simulink model "ACC_Scenario_006_cs"  (R2014b)
settings: Solver=ode5  SolverMode=SingleTasking  StartTime=0.0  StopTime=inf  FixedStep=1/100  RelTol=1e-3
PreLoadFcn:
  | mbxruntime.callbacks.PreLoadFcn(bdroot);
  | check_NUTS_defined;
  | 
  | assignin('base',['model_closed_' bdroot],false);addpath('../includes_ACC');
PostLoadFcn:
  | mbxruntime.callbacks.PostLoadFcn(bdroot);
InitFcn:
  | mbxruntime.callbacks.InitFcn(bdroot);
StartFcn:
  | mbxruntime.callbacks.StartFcn(bdroot);
StopFcn:
  | mbxruntime.callbacks.StopFcn(bdroot);
model workspace: external: MAT-File .\ACC_Scenario_006_cs_hws.mat (data not in the file)
undefined symbols (not defined in the file or in its folder): mbxruntime, OrientationPitch, OrientationRoll, PositionX, PositionY, PositionZ, tabledata, warningInitialVelocity, x0
undefined symbols (not defined in the file): ACC_Scenario_006_cs_061450488d6753c4, ACC_Scenario_006_cs_13896134c615b72a, ACC_Scenario_006_cs_18eaf2a52f2ef75d, ACC_Scenario_006_cs_59e375456829d2f0, ACC_Scenario_006_cs_8a2109b915871f11, ACC_Scenario_006_cs_a4f79cab717c06e2, ACC_Scenario_006_cs_Audi_A8_1_Dynamics_Simple_initialPitch, ACC_Scenario_006_cs_Audi_A8_1_Dynamics_Simple_initialRoll, ACC_Scenario_006_cs_Audi_A8_1_Dynamics_Simple_initialX, ACC_Scenario_006_cs_Audi_A8_1_Dynamics_Simple_initialY, ACC_Scenario_006_cs_Audi_A8_1_Dynamics_Simple_initialYaw, ACC_Scenario_006_cs_Audi_A8_1_Dynamics_Simple_initialZ, ACC_Scenario_006_cs_BMW_X5_1_Path_pathUniqueID, ACC_Scenario_006_cs_BMW_X5_1_SpeedProfile_speedProfileUniqueID, ACC_Scenario_006_cs_e4633c18fd34a832, ACC_Scenario_006_cs_f83c81dc10cd364a, ACC_Scenario_006_cs_Fiat_Bravo_1_Path_pathUniqueID, ACC_Scenario_006_cs_Ford_Fiesta_1_Path_pathUniqueID, ACC_Scenario_006_cs_Honda_Pan_European_1_Path_pathUniqueID, ACC_Scenario_006_cs_Mazda_RX8_1_Path_pathUniqueID, ACC_Scenario_006_cs_Sphere_1_Dynamics_Empty_STATE_Sphere_1_x0, ACC_Scenario_006_cs_Sphere_1_Dynamics_Empty_STATE_Sphere_1_y0, ACC_Scenario_006_cs_Sphere_1_Dynamics_Empty_STATE_Sphere_1_Yaw0, ACC_Scenario_006_cs_Sphere_1_Dynamics_Empty_STATE_Sphere_1_z0, ACC_Scenario_006_cs_Toyota_Yaris_1_Path_pathUniqueID, SteeringColumn, SteeringWheel, Wheel0, Wheel0_Suspension, Wheel1, Wheel1_Suspension, WheelL0, WheelL1, WheelR0, WheelR1
libraries: simulink_extras x60, simulink x21, PreScanSimulinkLibrary x5, PreScanUsefulBlocks x2
(part 1 of 24)
CloseFcn:
  | mbxruntime.callbacks.CloseFcn(bdroot);
  | evalin('base',['clear model_closed_' bdroot]);
settings Model: Creator=PRESCAN  LastModifiedBy=jenkins
settings DataIOCC: SignalLoggingSaveFormat=ModelDataLogs
settings OptimizationCC: InlineParams=on  ExpressionDepthLimit=2147483647  InitFltsAndDblsToZero=on
settings DebuggingCC: SaveWithParameterizedLinksMsg=none  UnderspecifiedInitializationDetection=Classic  MergeDetectMultiDrivingBlocksExec=none  SignalResolutionControl=TryResolveAllWithWarning  SolverPrmCheckMsg=none  MultiTaskDSMMsg=warning  MultiTaskCondExecSysMsg=none  FcnCallInpInsideContextMsg=UseLocalSettings  StateNameClashWarn=warning
settings ModelReferenceCC: UpdateModelReferenceTargets=IfOutOfDate
settings SFSimCC: SimParseCustomCode=off
settings SFSimCC: SimCustomHeaderCode=|
  | #include "prescan.h"
  | #include "prescan_platform.h"
settings RTWCC: IncludeERTFirstTime=on
settings GRTTargetCC: TargetFcnLib=ansi_tfl_tmw.mat  CombineOutputUpdateFcns=off  GRTInterface=on

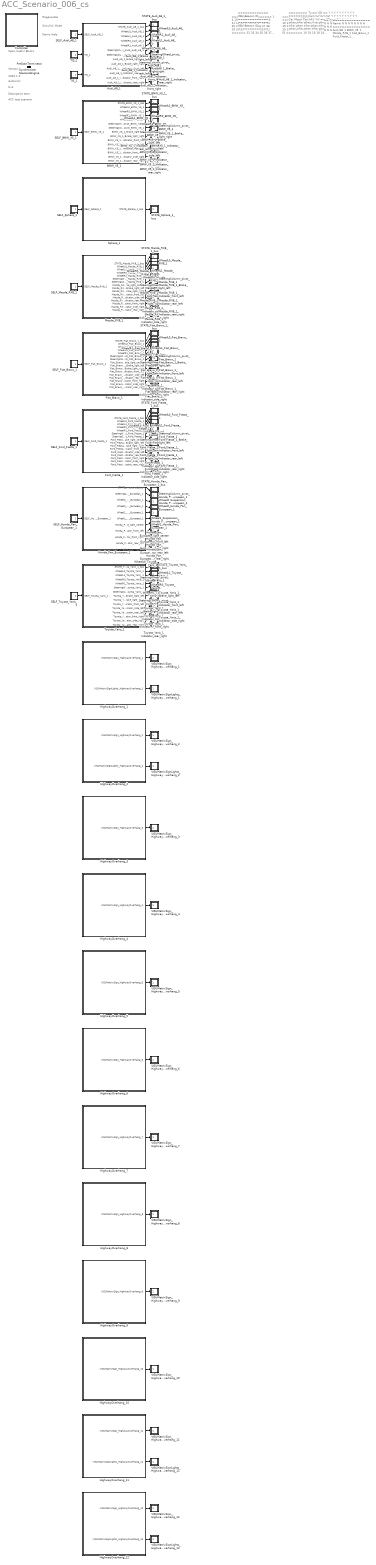
== system ACC_Scenario_006_cs ==
  note: Regenerate
  note: Simulink Mode
  note: Open Useful Blocks
  note: 2020.1.0
  note: Version:
  note: Author(s):
  note: N.A.
  note: Descriptive text:
  note: ACC test scenario
  note: Demo Help
  note: ======
      | Num ID
      | ======
      | 1
      | 4
      | 102
      | 231
      | 232
      | 233
      | 234
      | 8
      | 10
      | 11
      | 12
      | 13
      | 14
      | 15
      | 16
      | 17
      | 18
      | 19
      | 20
      | 21
      | 22
      | 23
      | 24
      | 25
      | 26
      | 27
      | 28
      | 29
      | 30
      | 31
      | ======
      | Num ID
      | ======
      | 32
      | 33
      | 34
      | 35
      | 36
      | 37
      | 38
      | 39
  note: =============
      | OBU-Beacon ID
      | =============
      |
      |
      |
      |
      |
      |
      |
      |
      |
      |
      |
      |
      |
      |
      |
      |
      |
      |
      |
      |
      |
      |
      |
      |
      |
      |
      |
      |
      |
      |
      | =============
      | OBU-Beacon ID
      | =============
  note: =======
      | Type ID
      | =======
      | 1
      | 1
      | 1
      | 1
      | 1
      | 2
      | 1
      | 19
      | 19
      | 19
      | 19
      | 19
      | 19
      | 19
      | 19
      | 19
      | 19
      | 19
      | 19
      | 19
      | 19
      | 19
      | 19
      | 19
      | 19
      | 19
      | 19
      | 19
      | 19
      | 19
      | =======
      | Type ID
      | =======
      | 19
      | 19
      | 19
      | 19
      | 19
      | 19
      | 19
      | 19
  note: ========
      | Type Tag
      | ========
      | Car
      | Car
      | Car
      | Car
      | Car
      | Motor
      | Car
      | Infra other
      | Infra other
      | Infra other
      | Infra other
      | Infra other
      | Infra other
      | Infra other
      | Infra other
      | Infra other
      | Infra other
      | Infra other
      | Infra other
      | Infra other
      | Infra other
      | Infra other
      | Infra other
      | Infra other
      | Infra other
      | Infra other
      | Infra other
      | Infra other
      | Infra other
      | Infra other
      | ========
      | Type Tag
      | ========
      | Infra other
      | Infra other
      | Infra other
      | Infra other
      | Infra other
      | Infra other
      | Infra other
      | Infra other
  note: ==
      | SD
      | ==
      | Y
      | Y
      | Y
      | Y
      | Y
      | Y
      | Y
      | Y
      | Y
      | Y
      | Y
      | Y
      | Y
      | Y
      | Y
      | Y
      | Y
      | Y
      | Y
      | Y
      | Y
      | Y
      | Y
      | Y
      | Y
      | Y
      | Y
      | Y
      | Y
      | Y
      | ==
      | SD
      | ==
      | Y
      | Y
      | Y
      | Y
      | Y
      | Y
      | Y
      | Y
  note: ==
      | CD
      | ==
      | N
      | N
      | N
      | N
      | N
      | N
      | N
      | N
      | N
      | N
      | N
      | N
      | N
      | N
      | N
      | N
      | N
      | N
      | N
      | N
      | N
      | N
      | N
      | N
      | N
      | N
      | N
      | N
      | N
      | N
      | ==
      | CD
      | ==
      | N
      | N
      | N
      | N
      | N
      | N
      | N
      | N
  note: ================
      | Name
      | ================
      | Audi_A8_1
      | BMW_X5_1
      | Mazda_RX8_1
      | Fiat_Bravo_1
      | Ford_Fiesta_1
      | Honda_Pan_European_1
      | Toyota_Yaris_1
      | ReflectorSign_1
      | ReflectorSign_2
      | ReflectorSign_3
      | ReflectorSign_4
      | ReflectorSign_5
      | ReflectorSign_6
      | ReflectorSign_7
      | ReflectorSign_8
      | ReflectorSign_9
      | ReflectorSign_10
      | ReflectorSign_11
      | ReflectorSign_12
      | ReflectorSign_13
      | ReflectorSign_14
      | ReflectorSign_15
      | ReflectorSign_16
      | ReflectorSign_17
      | ReflectorSign_18
      | ReflectorSign_19
      | ReflectorSign_20
      | ReflectorSign_21
      | ReflectorSign_22
      | ReflectorSign_23
      | ================
      | Name
      | ================
      | ReflectorSign_24
      | ReflectorSign_25
      | ReflectorSign_26
      | ReflectorSign_27
      | ReflectorSign_28
      | ReflectorSign_29
      | ReflectorSign_30
      | ReflectorSign_31
  Audi_A8_1 : Subsystem  Tag=WorldObjectSubSystem  InitFcn=UniqueId = '16';
      mask init:
      | modelPath = GenericModelHelper.getGenericModelFilePath('ModelDepo','Vehicles\Audi_A8\Audi_A8.pgmb','e33fe1ddcf3e8ae97caccbc8f2fa74ac');imagePath = GenericModelHelper.getCompilationPicture(modelPath, 'Audi_A8_HighPoly.png');
      mask Display: image(imread(imagePath));color('white');text(0, 0, ' ID=1\n')
  Audi_A8_1_Brake_light_left : Subsystem  Tag=actuator/BrakeLightL  Priority=0  LoadFcn=load('PreScanVisuLightActuatorData');load('PrescanRPYData');load('PrescanXYZData');load('PreScanRGBData')  mask(PreScan Sink Block: VisuActiveLight){}
      mask help:
      | The VisuActiveLight block provides a way for detailed animation of Light Sources, such as the indicator, brake, fog and main lights of a vehicle, or a light post.
      |
      | For more information, please click Help.
      settings: OpenFcn=open_system([gcb '/Actuator'],'mask')
      mask Help: eval('openHelp(209)')
      mask Display: image(imread('HeadLight.png'))
  Audi_A8_1_Brake_light_right : Subsystem  Tag=actuator/BrakeLightR  Priority=0  LoadFcn=load('PreScanVisuLightActuatorData');load('PrescanRPYData');load('PrescanXYZData');load('PreScanRGBData')  mask(PreScan Sink Block: VisuActiveLight){}
      mask help:
      | The VisuActiveLight block provides a way for detailed animation of Light Sources, such as the indicator, brake, fog and main lights of a vehicle, or a light post.
      |
      | For more information, please click Help.
      settings: OpenFcn=open_system([gcb '/Actuator'],'mask')
      mask Help: eval('openHelp(209)')
      mask Display: image(imread('HeadLight.png'))
  Audi_A8_1_Indicator_front_left : Subsystem  Tag=actuator/IndicatorFL  Priority=0  LoadFcn=load('PreScanVisuLightActuatorData');load('PrescanRPYData');load('PrescanXYZData');load('PreScanRGBData')  mask(PreScan Sink Block: VisuActiveLight){}
      mask help:
      | The VisuActiveLight block provides a way for detailed animation of Light Sources, such as the indicator, brake, fog and main lights of a vehicle, or a light post.
      |
      | For more information, please click Help.
      settings: OpenFcn=open_system([gcb '/Actuator'],'mask')
      mask Help: eval('openHelp(209)')
      mask Display: image(imread('HeadLight.png'))
  Audi_A8_1_Indicator_front_right : Subsystem  Tag=actuator/IndicatorFR  Priority=0  LoadFcn=load('PreScanVisuLightActuatorData');load('PrescanRPYData');load('PrescanXYZData');load('PreScanRGBData')  mask(PreScan Sink Block: VisuActiveLight){}
      mask help:
      | The VisuActiveLight block provides a way for detailed animation of Light Sources, such as the indicator, brake, fog and main lights of a vehicle, or a light post.
      |
      | For more information, please click Help.
      settings: OpenFcn=open_system([gcb '/Actuator'],'mask')
      mask Help: eval('openHelp(209)')
      mask Display: image(imread('HeadLight.png'))
  Audi_A8_1_Indicator_rear_left : Subsystem  Tag=actuator/IndicatorRL  Priority=0  LoadFcn=load('PreScanVisuLightActuatorData');load('PrescanRPYData');load('PrescanXYZData');load('PreScanRGBData')  mask(PreScan Sink Block: VisuActiveLight){}
      mask help:
      | The VisuActiveLight block provides a way for detailed animation of Light Sources, such as the indicator, brake, fog and main lights of a vehicle, or a light post.
      |
      | For more information, please click Help.
      settings: OpenFcn=open_system([gcb '/Actuator'],'mask')
      mask Help: eval('openHelp(209)')
      mask Display: image(imread('HeadLight.png'))
  Audi_A8_1_Indicator_rear_right : Subsystem  Tag=actuator/IndicatorRR  Priority=0  LoadFcn=load('PreScanVisuLightActuatorData');load('PrescanRPYData');load('PrescanXYZData');load('PreScanRGBData')  mask(PreScan Sink Block: VisuActiveLight){}
      mask help:
      | The VisuActiveLight block provides a way for detailed animation of Light Sources, such as the indicator, brake, fog and main lights of a vehicle, or a light post.
      |
      | For more information, please click Help.
      settings: OpenFcn=open_system([gcb '/Actuator'],'mask')
      mask Help: eval('openHelp(209)')
      mask Display: image(imread('HeadLight.png'))
  BMW_X5_1 : Subsystem  Tag=WorldObjectSubSystem  InitFcn=UniqueId = '21';
      mask init:
      | modelPath = GenericModelHelper.getGenericModelFilePath('ModelDepo','Vehicles\BMW_X5\BMW_X5.pgmb','bfeb1c11467705ab888b3011684c848b');imagePath = GenericModelHelper.getCompilationPicture(modelPath, 'BMW_X5_HighPoly.png');
      mask Display: image(imread(imagePath));color('white');text(0, 0, ' ID=4\n')
  BMW_X5_1_Brake_light_left : Subsystem  Tag=actuator/BrakeLightL  Priority=0  LoadFcn=load('PreScanVisuLightActuatorData');load('PrescanRPYData');load('PrescanXYZData');load('PreScanRGBData')  mask(PreScan Sink Block: VisuActiveLight){}
      mask help:
      | The VisuActiveLight block provides a way for detailed animation of Light Sources, such as the indicator, brake, fog and main lights of a vehicle, or a light post.
      |
      | For more information, please click Help.
      settings: OpenFcn=open_system([gcb '/Actuator'],'mask')
      mask Help: eval('openHelp(209)')
      mask Display: image(imread('HeadLight.png'))
  BMW_X5_1_Brake_light_right : Subsystem  Tag=actuator/BrakeLightR  Priority=0  LoadFcn=load('PreScanVisuLightActuatorData');load('PrescanRPYData');load('PrescanXYZData');load('PreScanRGBData')  mask(PreScan Sink Block: VisuActiveLight){}
      mask help:
      | The VisuActiveLight block provides a way for detailed animation of Light Sources, such as the indicator, brake, fog and main lights of a vehicle, or a light post.
      |
      | For more information, please click Help.
      settings: OpenFcn=open_system([gcb '/Actuator'],'mask')
      mask Help: eval('openHelp(209)')
      mask Display: image(imread('HeadLight.png'))
  BMW_X5_1_Indicator_front_left : Subsystem  Tag=actuator/IndicatorFL  Priority=0  LoadFcn=load('PreScanVisuLightActuatorData');load('PrescanRPYData');load('PrescanXYZData');load('PreScanRGBData')  mask(PreScan Sink Block: VisuActiveLight){}
      mask help:
      | The VisuActiveLight block provides a way for detailed animation of Light Sources, such as the indicator, brake, fog and main lights of a vehicle, or a light post.
      |
      | For more information, please click Help.
      settings: OpenFcn=open_system([gcb '/Actuator'],'mask')
      mask Help: eval('openHelp(209)')
      mask Display: image(imread('HeadLight.png'))
  BMW_X5_1_Indicator_front_right : Subsystem  Tag=actuator/IndicatorFR  Priority=0  LoadFcn=load('PreScanVisuLightActuatorData');load('PrescanRPYData');load('PrescanXYZData');load('PreScanRGBData')  mask(PreScan Sink Block: VisuActiveLight){}
      mask help:
      | The VisuActiveLight block provides a way for detailed animation of Light Sources, such as the indicator, brake, fog and main lights of a vehicle, or a light post.
      |
      | For more information, please click Help.
      settings: OpenFcn=open_system([gcb '/Actuator'],'mask')
      mask Help: eval('openHelp(209)')
      mask Display: image(imread('HeadLight.png'))
  BMW_X5_1_Indicator_rear_left : Subsystem  Tag=actuator/IndicatorRL  Priority=0  LoadFcn=load('PreScanVisuLightActuatorData');load('PrescanRPYData');load('PrescanXYZData');load('PreScanRGBData')  mask(PreScan Sink Block: VisuActiveLight){}
      mask help:
      | The VisuActiveLight block provides a way for detailed animation of Light Sources, such as the indicator, brake, fog and main lights of a vehicle, or a light post.
      |
      | For more information, please click Help.
      settings: OpenFcn=open_system([gcb '/Actuator'],'mask')
      mask Help: eval('openHelp(209)')
      mask Display: image(imread('HeadLight.png'))
  BMW_X5_1_Indicator_rear_right : Subsystem  Tag=actuator/IndicatorRR  Priority=0  LoadFcn=load('PreScanVisuLightActuatorData');load('PrescanRPYData');load('PrescanXYZData');load('PreScanRGBData')  mask(PreScan Sink Block: VisuActiveLight){}
      mask help:
      | The VisuActiveLight block provides a way for detailed animation of Light Sources, such as the indicator, brake, fog and main lights of a vehicle, or a light post.
      |
      | For more information, please click Help.
      settings: OpenFcn=open_system([gcb '/Actuator'],'mask')
      mask Help: eval('openHelp(209)')
      mask Display: image(imread('HeadLight.png'))
  BMW_X5_1_Indicator_side_left : Subsystem  Tag=actuator/IndicatorSL  Priority=0  LoadFcn=load('PreScanVisuLightActuatorData');load('PrescanRPYData');load('PrescanXYZData');load('PreScanRGBData')  mask(PreScan Sink Block: VisuActiveLight){}
      mask help:
      | The VisuActiveLight block provides a way for detailed animation of Light Sources, such as the indicator, brake, fog and main lights of a vehicle, or a light post.
      |
      | For more information, please click Help.
      settings: OpenFcn=open_system([gcb '/Actuator'],'mask')
      mask Help: eval('openHelp(209)')
      mask Display: image(imread('HeadLight.png'))
  BMW_X5_1_Indicator_side_right : Subsystem  Tag=actuator/IndicatorSR  Priority=0  LoadFcn=load('PreScanVisuLightActuatorData');load('PrescanRPYData');load('PrescanXYZData');load('PreScanRGBData')  mask(PreScan Sink Block: VisuActiveLight){}
      mask help:
      | The VisuActiveLight block provides a way for detailed animation of Light Sources, such as the indicator, brake, fog and main lights of a vehicle, or a light post.
      |
      | For more information, please click Help.
      settings: OpenFcn=open_system([gcb '/Actuator'],'mask')
      mask Help: eval('openHelp(209)')
      mask Display: image(imread('HeadLight.png'))
  Controller : Subsystem  Description=8A3CD2955739A82C886C20AE3E253D78460D53180EE2C1B14CC08DF75A70BE77  Priority=-1  LoadFcn=load PreScanControllerData  mask(PreScan Simulation Controller){prescanversion='2020.1.0', ModelReferencing=off, TimeStep=1/100, ControlMode=0, PreScanExecutionMode=on, ControllerCount=0, ControllerIndex=0, ControllerOptions=''}
      mask prompts: prescanversion "PreScan Version"; ModelReferencing "Use Model Referencing"; TimeStep "Upload Period [s]"; ControlMode "Control Mode"; PreScanExecutionMode "Execution Mode"; ControllerCount "Controller Count"; ControllerIndex "Controller Index"; ControllerOptions "Controller Options"
      mask help:
      | Please do not remove this block from the compilation sheet,
      | as it connects the model to the PreScan environment.
      mask init:
      | model = bdroot(gcb);
      | ExperimentFile = mbxruntime.findExperimentFile(model,true); %relative path
      | 
      | [d1, d2, d3, prescandata] = prescan_Settings();
      | ModelDepo = fullfile(prescandata,'ModelDepo'); 
      | 
      | RTmode = mbxruntime.getRTMode(model);
      | 
      | SimulationMode = get_param(bdroot,'SimulationMode');
      | if strcmp(SimulationMode, 'rapid-accelerator')
      |     SimulationMode = 'external';
      | end
      | TargetName = get_param(bdroot,'SystemTargetFile');
      settings: ModelCloseFcn=assignin('base',['model_closed_' bdroot],true);
      mask Help: eval('openHelp(812)')
      mask Display: image(imread('prescanlogo.ico'))
  Fiat_Bravo_1 : Subsystem  Tag=WorldObjectSubSystem  InitFcn=UniqueId = '350';
      mask init:
      | modelPath = GenericModelHelper.getGenericModelFilePath('ModelDepo','Vehicles\Fiat_Bravo\Fiat_Bravo.pgmb','a97eb0ec4093646e5d079d2ab9a2eab7');imagePath = GenericModelHelper.getCompilationPicture(modelPath, 'Fiat_Bravo_HighPoly.png');
      mask Display: image(imread(imagePath));color('white');text(0, 0, ' ID=231\n')
  Fiat_Bravo_1_Brake_light_center : Subsystem  Tag=actuator/BrakeLightM  Priority=0  LoadFcn=load('PreScanVisuLightActuatorData');load('PrescanRPYData');load('PrescanXYZData');load('PreScanRGBData')  mask(PreScan Sink Block: VisuActiveLight){}
      mask help:
      | The VisuActiveLight block provides a way for detailed animation of Light Sources, such as the indicator, brake, fog and main lights of a vehicle, or a light post.
      |
      | For more information, please click Help.
      settings: OpenFcn=open_system([gcb '/Actuator'],'mask')
      mask Help: eval('openHelp(209)')
      mask Display: image(imread('HeadLight.png'))
  Fiat_Bravo_1_Brake_light_left : Subsystem  Tag=actuator/BrakeLightL  Priority=0  LoadFcn=load('PreScanVisuLightActuatorData');load('PrescanRPYData');load('PrescanXYZData');load('PreScanRGBData')  mask(PreScan Sink Block: VisuActiveLight){}
      mask help:
      | The VisuActiveLight block provides a way for detailed animation of Light Sources, such as the indicator, brake, fog and main lights of a vehicle, or a light post.
      |
      | For more information, please click Help.
      settings: OpenFcn=open_system([gcb '/Actuator'],'mask')
      mask Help: eval('openHelp(209)')
      mask Display: image(imread('HeadLight.png'))
  Fiat_Bravo_1_Brake_light_right : Subsystem  Tag=actuator/BrakeLightR  Priority=0  LoadFcn=load('PreScanVisuLightActuatorData');load('PrescanRPYData');load('PrescanXYZData');load('PreScanRGBData')  mask(PreScan Sink Block: VisuActiveLight){}
      mask help:
      | The VisuActiveLight block provides a way for detailed animation of Light Sources, such as the indicator, brake, fog and main lights of a vehicle, or a light post.
      |
      | For more information, please click Help.
      settings: OpenFcn=open_system([gcb '/Actuator'],'mask')
      mask Help: eval('openHelp(209)')
      mask Display: image(imread('HeadLight.png'))
  Fiat_Bravo_1_Indicator_front_left : Subsystem  Tag=actuator/IndicatorFL  Priority=0  LoadFcn=load('PreScanVisuLightActuatorData');load('PrescanRPYData');load('PrescanXYZData');load('PreScanRGBData')  mask(PreScan Sink Block: VisuActiveLight){}
      mask help:
      | The VisuActiveLight block provides a way for detailed animation of Light Sources, such as the indicator, brake, fog and main lights of a vehicle, or a light post.
      |
      | For more information, please click Help.
      settings: OpenFcn=open_system([gcb '/Actuator'],'mask')
      mask Help: eval('openHelp(209)')
      mask Display: image(imread('HeadLight.png'))
  Fiat_Bravo_1_Indicator_front_right : Subsystem  Tag=actuator/IndicatorFR  Priority=0  LoadFcn=load('PreScanVisuLightActuatorData');load('PrescanRPYData');load('PrescanXYZData');load('PreScanRGBData')  mask(PreScan Sink Block: VisuActiveLight){}
      mask help:
      | The VisuActiveLight block provides a way for detailed animation of Light Sources, such as the indicator, brake, fog and main lights of a vehicle, or a light post.
      |
      | For more information, please click Help.
      settings: OpenFcn=open_system([gcb '/Actuator'],'mask')
      mask Help: eval('openHelp(209)')
      mask Display: image(imread('HeadLight.png'))
  Fiat_Bravo_1_Indicator_rear_left : Subsystem  Tag=actuator/IndicatorRL  Priority=0  LoadFcn=load('PreScanVisuLightActuatorData');load('PrescanRPYData');load('PrescanXYZData');load('PreScanRGBData')  mask(PreScan Sink Block: VisuActiveLight){}
      mask help:
      | The VisuActiveLight block provides a way for detailed animation of Light Sources, such as the indicator, brake, fog and main lights of a vehicle, or a light post.
      |
      | For more information, please click Help.
      settings: OpenFcn=open_system([gcb '/Actuator'],'mask')
      mask Help: eval('openHelp(209)')
      mask Display: image(imread('HeadLight.png'))
  Fiat_Bravo_1_Indicator_rear_right : Subsystem  Tag=actuator/IndicatorRR  Priority=0  LoadFcn=load('PreScanVisuLightActuatorData');load('PrescanRPYData');load('PrescanXYZData');load('PreScanRGBData')  mask(PreScan Sink Block: VisuActiveLight){}
      mask help:
      | The VisuActiveLight block provides a way for detailed animation of Light Sources, such as the indicator, brake, fog and main lights of a vehicle, or a light post.
      |
      | For more information, please click Help.
      settings: OpenFcn=open_system([gcb '/Actuator'],'mask')
      mask Help: eval('openHelp(209)')
      mask Display: image(imread('HeadLight.png'))
  Fiat_Bravo_1_Indicator_side_left : Subsystem  Tag=actuator/IndicatorSL  Priority=0  LoadFcn=load('PreScanVisuLightActuatorData');load('PrescanRPYData');load('PrescanXYZData');load('PreScanRGBData')  mask(PreScan Sink Block: VisuActiveLight){}
      mask help:
      | The VisuActiveLight block provides a way for detailed animation of Light Sources, such as the indicator, brake, fog and main lights of a vehicle, or a light post.
      |
      | For more information, please click Help.
      settings: OpenFcn=open_system([gcb '/Actuator'],'mask')
      mask Help: eval('openHelp(209)')
      mask Display: image(imread('HeadLight.png'))
  Fiat_Bravo_1_Indicator_side_right : Subsystem  Tag=actuator/IndicatorSR  Priority=0  LoadFcn=load('PreScanVisuLightActuatorData');load('PrescanRPYData');load('PrescanXYZData');load('PreScanRGBData')  mask(PreScan Sink Block: VisuActiveLight){}
      mask help:
      | The VisuActiveLight block provides a way for detailed animation of Light Sources, such as the indicator, brake, fog and main lights of a vehicle, or a light post.
      |
      | For more information, please click Help.
      settings: OpenFcn=open_system([gcb '/Actuator'],'mask')
      mask Help: eval('openHelp(209)')
      mask Display: image(imread('HeadLight.png'))
  Ford_Fiesta_1 : Subsystem  Tag=WorldObjectSubSystem  InitFcn=UniqueId = '353';
      mask init:
      | modelPath = GenericModelHelper.getGenericModelFilePath('ModelDepo','Vehicles\Ford_Fiesta\Ford_Fiesta.pgmb','fe2c7a73e0a60cba76689b71cd1bb76a');imagePath = GenericModelHelper.getCompilationPicture(modelPath, 'Ford_Fiesta_HighPoly.png');
      mask Display: image(imread(imagePath));color('white');text(0, 0, ' ID=232\n')
  Ford_Fiesta_1_Brake_light_center : Subsystem  Tag=actuator/BrakeLightM  Priority=0  LoadFcn=load('PreScanVisuLightActuatorData');load('PrescanRPYData');load('PrescanXYZData');load('PreScanRGBData')  mask(PreScan Sink Block: VisuActiveLight){}
      mask help:
      | The VisuActiveLight block provides a way for detailed animation of Light Sources, such as the indicator, brake, fog and main lights of a vehicle, or a light post.
      |
      | For more information, please click Help.
      settings: OpenFcn=open_system([gcb '/Actuator'],'mask')
      mask Help: eval('openHelp(209)')
      mask Display: image(imread('HeadLight.png'))
  Ford_Fiesta_1_Brake_light_left : Subsystem  Tag=actuator/BrakeLightL  Priority=0  LoadFcn=load('PreScanVisuLightActuatorData');load('PrescanRPYData');load('PrescanXYZData');load('PreScanRGBData')  mask(PreScan Sink Block: VisuActiveLight){}
      mask help:
      | The VisuActiveLight block provides a way for detailed animation of Light Sources, such as the indicator, brake, fog and main lights of a vehicle, or a light post.
      |
      | For more information, please click Help.
      settings: OpenFcn=open_system([gcb '/Actuator'],'mask')
      mask Help: eval('openHelp(209)')
      mask Display: image(imread('HeadLight.png'))
  Ford_Fiesta_1_Brake_light_right : Subsystem  Tag=actuator/BrakeLightR  Priority=0  LoadFcn=load('PreScanVisuLightActuatorData');load('PrescanRPYData');load('PrescanXYZData');load('PreScanRGBData')  mask(PreScan Sink Block: VisuActiveLight){}
      mask help:
      | The VisuActiveLight block provides a way for detailed animation of Light Sources, such as the indicator, brake, fog and main lights of a vehicle, or a light post.
      |
      | For more information, please click Help.
      settings: OpenFcn=open_system([gcb '/Actuator'],'mask')
      mask Help: eval('openHelp(209)')
      mask Display: image(imread('HeadLight.png'))
  Ford_Fiesta_1_Indicator_front_left : Subsystem  Tag=actuator/IndicatorFL  Priority=0  LoadFcn=load('PreScanVisuLightActuatorData');load('PrescanRPYData');load('PrescanXYZData');load('PreScanRGBData')  mask(PreScan Sink Block: VisuActiveLight){}
      mask help:
      | The VisuActiveLight block provides a way for detailed animation of Light Sources, such as the indicator, brake, fog and main lights of a vehicle, or a light post.
      |
      | For more information, please click Help.
      settings: OpenFcn=open_system([gcb '/Actuator'],'mask')
      mask Help: eval('openHelp(209)')
      mask Display: image(imread('HeadLight.png'))
  Ford_Fiesta_1_Indicator_front_right : Subsystem  Tag=actuator/IndicatorFR  Priority=0  LoadFcn=load('PreScanVisuLightActuatorData');load('PrescanRPYData');load('PrescanXYZData');load('PreScanRGBData')  mask(PreScan Sink Block: VisuActiveLight){}
      mask help:
      | The VisuActiveLight block provides a way for detailed animation of Light Sources, such as the indicator, brake, fog and main lights of a vehicle, or a light post.
      |
      | For more information, please click Help.
      settings: OpenFcn=open_system([gcb '/Actuator'],'mask')
      mask Help: eval('openHelp(209)')
      mask Display: image(imread('HeadLight.png'))
  Ford_Fiesta_1_Indicator_rear_left : Subsystem  Tag=actuator/IndicatorRL  Priority=0  LoadFcn=load('PreScanVisuLightActuatorData');load('PrescanRPYData');load('PrescanXYZData');load('PreScanRGBData')  mask(PreScan Sink Block: VisuActiveLight){}
      mask help:
      | The VisuActiveLight block provides a way for detailed animation of Light Sources, such as the indicator, brake, fog and main lights of a vehicle, or a light post.
      |
      | For more information, please click Help.
      settings: OpenFcn=open_system([gcb '/Actuator'],'mask')
      mask Help: eval('openHelp(209)')
      mask Display: image(imread('HeadLight.png'))
  Ford_Fiesta_1_Indicator_rear_right : Subsystem  Tag=actuator/IndicatorRR  Priority=0  LoadFcn=load('PreScanVisuLightActuatorData');load('PrescanRPYData');load('PrescanXYZData');load('PreScanRGBData')  mask(PreScan Sink Block: VisuActiveLight){}
      mask help:
      | The VisuActiveLight block provides a way for detailed animation of Light Sources, such as the indicator, brake, fog and main lights of a vehicle, or a light post.
      |
      | For more information, please click Help.
      settings: OpenFcn=open_system([gcb '/Actuator'],'mask')
      mask Help: eval('openHelp(209)')
      mask Display: image(imread('HeadLight.png'))
  Ford_Fiesta_1_Indicator_side_left : Subsystem  Tag=actuator/IndicatorSL  Priority=0  LoadFcn=load('PreScanVisuLightActuatorData');load('PrescanRPYData');load('PrescanXYZData');load('PreScanRGBData')  mask(PreScan Sink Block: VisuActiveLight){}
      mask help:
      | The VisuActiveLight block provides a way for detailed animation of Light Sources, such as the indicator, brake, fog and main lights of a vehicle, or a light post.
      |
      | For more information, please click Help.
      settings: OpenFcn=open_system([gcb '/Actuator'],'mask')
      mask Help: eval('openHelp(209)')
      mask Display: image(imread('HeadLight.png'))
  Ford_Fiesta_1_Indicator_side_right : Subsystem  Tag=actuator/IndicatorSR  Priority=0  LoadFcn=load('PreScanVisuLightActuatorData');load('PrescanRPYData');load('PrescanXYZData');load('PreScanRGBData')  mask(PreScan Sink Block: VisuActiveLight){}
      mask help:
      | The VisuActiveLight block provides a way for detailed animation of Light Sources, such as the indicator, brake, fog and main lights of a vehicle, or a light post.
      |
      | For more information, please click Help.
      settings: OpenFcn=open_system([gcb '/Actuator'],'mask')
      mask Help: eval('openHelp(209)')
      mask Display: image(imread('HeadLight.png'))
  HighwayOverhang_1 : Subsystem  Tag=WorldObjectSubSystem  InitFcn=UniqueId = '109';
      mask init:
      | imagePath=which('HighwayOverhang.jpg');
      mask Display: image(imread(imagePath));color('white');text(0, 0, ' ID=88\n')
  HighwayOverhang_10 : Subsystem  Tag=WorldObjectSubSystem  InitFcn=UniqueId = '119';
      mask init:
      | imagePath=which('HighwayOverhang.jpg');
      mask Display: image(imread(imagePath));color('white');text(0, 0, ' ID=99\n')
  HighwayOverhang_11 : Subsystem  Tag=WorldObjectSubSystem  InitFcn=UniqueId = '120';
      mask init:
      | imagePath=which('HighwayOverhang.jpg');
      mask Display: image(imread(imagePath));color('white');text(0, 0, ' ID=100\n')
  HighwayOverhang_12 : Subsystem  Tag=WorldObjectSubSystem  InitFcn=UniqueId = '121';
      mask init:
      | imagePath=which('HighwayOverhang.jpg');
      mask Display: image(imread(imagePath));color('white');text(0, 0, ' ID=101\n')
  HighwayOverhang_2 : Subsystem  Tag=WorldObjectSubSystem  InitFcn=UniqueId = '110';
      mask init:
      | imagePath=which('HighwayOverhang.jpg');
      mask Display: image(imread(imagePath));color('white');text(0, 0, ' ID=90\n')
  HighwayOverhang_3 : Subsystem  Tag=WorldObjectSubSystem  InitFcn=UniqueId = '112';
      mask init:
      | imagePath=which('HighwayOverhang.jpg');
      mask Display: image(imread(imagePath));color('white');text(0, 0, ' ID=89\n')
  HighwayOverhang_4 : Subsystem  Tag=WorldObjectSubSystem  InitFcn=UniqueId = '113';
      mask init:
      | imagePath=which('HighwayOverhang.jpg');
      mask Display: image(imread(imagePath));color('white');text(0, 0, ' ID=93\n')
  HighwayOverhang_5 : Subsystem  Tag=WorldObjectSubSystem  InitFcn=UniqueId = '114';
      mask init:
      | imagePath=which('HighwayOverhang.jpg');
      mask Display: image(imread(imagePath));color('white');text(0, 0, ' ID=92\n')
  HighwayOverhang_6 : Subsystem  Tag=WorldObjectSubSystem  InitFcn=UniqueId = '115';
      mask init:
      | imagePath=which('HighwayOverhang.jpg');
      mask Display: image(imread(imagePath));color('white');text(0, 0, ' ID=95\n')
  HighwayOverhang_7 : Subsystem  Tag=WorldObjectSubSystem  InitFcn=UniqueId = '116';
      mask init:
      | imagePath=which('HighwayOverhang.jpg');
      mask Display: image(imread(imagePath));color('white');text(0, 0, ' ID=94\n')
  HighwayOverhang_8 : Subsystem  Tag=WorldObjectSubSystem  InitFcn=UniqueId = '117';
      mask init:
      | imagePath=which('HighwayOverhang.jpg');
      mask Display: image(imread(imagePath));color('white');text(0, 0, ' ID=97\n')
  HighwayOverhang_9 : Subsystem  Tag=WorldObjectSubSystem  InitFcn=UniqueId = '118';
      mask init:
      | imagePath=which('HighwayOverhang.jpg');
      mask Display: image(imread(imagePath));color('white');text(0, 0, ' ID=98\n')
  Honda_Pan_European_1 : Subsystem  Tag=WorldObjectSubSystem  InitFcn=UniqueId = '356';
      mask init:
      | modelPath = GenericModelHelper.getGenericModelFilePath('ModelDepo','Vehicles\Honda_Pan_European_With_Driver\Honda_Pan_European_With_Driver.pgmb','87ba31455683eb3e7a0d63db23b59554');imagePath = GenericModelHelper.getCompilationPicture(modelPath, 'Honda_Pan_European_HighPoly_With_Driver.png');
      mask Display: image(imread(imagePath));color('white');text(0, 0, ' ID=233\n')
  Honda_Pan_European_1_Brake_light_center : Subsystem  Tag=actuator/BrakeLightM  Priority=0  LoadFcn=load('PreScanVisuLightActuatorData');load('PrescanRPYData');load('PrescanXYZData');load('PreScanRGBData')  mask(PreScan Sink Block: VisuActiveLight){}
      mask help:
      | The VisuActiveLight block provides a way for detailed animation of Light Sources, such as the indicator, brake, fog and main lights of a vehicle, or a light post.
      |
      | For more information, please click Help.
      settings: OpenFcn=open_system([gcb '/Actuator'],'mask')
      mask Help: eval('openHelp(209)')
      mask Display: image(imread('HeadLight.png'))
  Honda_Pan_European_1_Indicator_front_left : Subsystem  Tag=actuator/IndicatorFL  Priority=0  LoadFcn=load('PreScanVisuLightActuatorData');load('PrescanRPYData');load('PrescanXYZData');load('PreScanRGBData')  mask(PreScan Sink Block: VisuActiveLight){}
      mask help:
      | The VisuActiveLight block provides a way for detailed animation of Light Sources, such as the indicator, brake, fog and main lights of a vehicle, or a light post.
      |
      | For more information, please click Help.
      settings: OpenFcn=open_system([gcb '/Actuator'],'mask')
      mask Help: eval('openHelp(209)')
      mask Display: image(imread('HeadLight.png'))
  Honda_Pan_European_1_Indicator_front_right : Subsystem  Tag=actuator/IndicatorFR  Priority=0  LoadFcn=load('PreScanVisuLightActuatorData');load('PrescanRPYData');load('PrescanXYZData');load('PreScanRGBData')  mask(PreScan Sink Block: VisuActiveLight){}
      mask help:
      | The VisuActiveLight block provides a way for detailed animation of Light Sources, such as the indicator, brake, fog and main lights of a vehicle, or a light post.
      |
      | For more information, please click Help.
      settings: OpenFcn=open_system([gcb '/Actuator'],'mask')
      mask Help: eval('openHelp(209)')
      mask Display: image(imread('HeadLight.png'))
  Honda_Pan_European_1_Indicator_rear_left : Subsystem  Tag=actuator/IndicatorRL  Priority=0  LoadFcn=load('PreScanVisuLightActuatorData');load('PrescanRPYData');load('PrescanXYZData');load('PreScanRGBData')  mask(PreScan Sink Block: VisuActiveLight){}
      mask help:
      | The VisuActiveLight block provides a way for detailed animation of Light Sources, such as the indicator, brake, fog and main lights of a vehicle, or a light post.
      |
      | For more information, please click Help.
      settings: OpenFcn=open_system([gcb '/Actuator'],'mask')
      mask Help: eval('openHelp(209)')
      mask Display: image(imread('HeadLight.png'))
  Honda_Pan_European_1_Indicator_rear_right : Subsystem  Tag=actuator/IndicatorRR  Priority=0  LoadFcn=load('PreScanVisuLightActuatorData');load('PrescanRPYData');load('PrescanXYZData');load('PreScanRGBData')  mask(PreScan Sink Block: VisuActiveLight){}
      mask help:
      | The VisuActiveLight block provides a way for detailed animation of Light Sources, such as the indicator, brake, fog and main lights of a vehicle, or a light post.
      |
      | For more information, please click Help.
      settings: OpenFcn=open_system([gcb '/Actuator'],'mask')
      mask Help: eval('openHelp(209)')
      mask Display: image(imread('HeadLight.png'))
  Mazda_RX8_1 : Subsystem  Tag=WorldObjectSubSystem  InitFcn=UniqueId = '345';
      mask init:
      | modelPath = GenericModelHelper.getGenericModelFilePath('ModelDepo','Vehicles\Mazda_RX8\Mazda_RX8.pgmb','1e55a2e40efa576b7f4fb93bae35d605');imagePath = GenericModelHelper.getCompilationPicture(modelPath, 'Mazda_RX8_HighPoly.png');
      mask Display: image(imread(imagePath));color('white');text(0, 0, ' ID=102\n')
  Mazda_RX8_1_Brake_light_center : Subsystem  Tag=actuator/BrakeLightM  Priority=0  LoadFcn=load('PreScanVisuLightActuatorData');load('PrescanRPYData');load('PrescanXYZData');load('PreScanRGBData')  mask(PreScan Sink Block: VisuActiveLight){}
      mask help:
      | The VisuActiveLight block provides a way for detailed animation of Light Sources, such as the indicator, brake, fog and main lights of a vehicle, or a light post.
      |
      | For more information, please click Help.
      settings: OpenFcn=open_system([gcb '/Actuator'],'mask')
      mask Help: eval('openHelp(209)')
      mask Display: image(imread('HeadLight.png'))
  Mazda_RX8_1_Brake_light_left : Subsystem  Tag=actuator/BrakeLightL  Priority=0  LoadFcn=load('PreScanVisuLightActuatorData');load('PrescanRPYData');load('PrescanXYZData');load('PreScanRGBData')  mask(PreScan Sink Block: VisuActiveLight){}
      mask help:
      | The VisuActiveLight block provides a way for detailed animation of Light Sources, such as the indicator, brake, fog and main lights of a vehicle, or a light post.
      |
      | For more information, please click Help.
      settings: OpenFcn=open_system([gcb '/Actuator'],'mask')
      mask Help: eval('openHelp(209)')
      mask Display: image(imread('HeadLight.png'))
  Mazda_RX8_1_Brake_light_right : Subsystem  Tag=actuator/BrakeLightR  Priority=0  LoadFcn=load('PreScanVisuLightActuatorData');load('PrescanRPYData');load('PrescanXYZData');load('PreScanRGBData')  mask(PreScan Sink Block: VisuActiveLight){}
      mask help:
      | The VisuActiveLight block provides a way for detailed animation of Light Sources, such as the indicator, brake, fog and main lights of a vehicle, or a light post.
      |
      | For more information, please click Help.
      settings: OpenFcn=open_system([gcb '/Actuator'],'mask')
      mask Help: eval('openHelp(209)')
      mask Display: image(imread('HeadLight.png'))
  Mazda_RX8_1_Indicator_front_left : Subsystem  Tag=actuator/IndicatorFL  Priority=0  LoadFcn=load('PreScanVisuLightActuatorData');load('PrescanRPYData');load('PrescanXYZData');load('PreScanRGBData')  mask(PreScan Sink Block: VisuActiveLight){}
      mask help:
      | The VisuActiveLight block provides a way for detailed animation of Light Sources, such as the indicator, brake, fog and main lights of a vehicle, or a light post.
      |
      | For more information, please click Help.
      settings: OpenFcn=open_system([gcb '/Actuator'],'mask')
      mask Help: eval('openHelp(209)')
      mask Display: image(imread('HeadLight.png'))
  Mazda_RX8_1_Indicator_front_right : Subsystem  Tag=actuator/IndicatorFR  Priority=0  LoadFcn=load('PreScanVisuLightActuatorData');load('PrescanRPYData');load('PrescanXYZData');load('PreScanRGBData')  mask(PreScan Sink Block: VisuActiveLight){}
      mask help:
      | The VisuActiveLight block provides a way for detailed animation of Light Sources, such as the indicator, brake, fog and main lights of a vehicle, or a light post.
      |
      | For more information, please click Help.
      settings: OpenFcn=open_system([gcb '/Actuator'],'mask')
      mask Help: eval('openHelp(209)')
      mask Display: image(imread('HeadLight.png'))
  Mazda_RX8_1_Indicator_rear_left : Subsystem  Tag=actuator/IndicatorRL  Priority=0  LoadFcn=load('PreScanVisuLightActuatorData');load('PrescanRPYData');load('PrescanXYZData');load('PreScanRGBData')  mask(PreScan Sink Block: VisuActiveLight){}
      mask help:
      | The VisuActiveLight block provides a way for detailed animation of Light Sources, such as the indicator, brake, fog and main lights of a vehicle, or a light post.
      |
      | For more information, please click Help.
      settings: OpenFcn=open_system([gcb '/Actuator'],'mask')
      mask Help: eval('openHelp(209)')
      mask Display: image(imread('HeadLight.png'))
  Mazda_RX8_1_Indicator_rear_right : Subsystem  Tag=actuator/IndicatorRR  Priority=0  LoadFcn=load('PreScanVisuLightActuatorData');load('PrescanRPYData');load('PrescanXYZData');load('PreScanRGBData')  mask(PreScan Sink Block: VisuActiveLight){}
      mask help:
      | The VisuActiveLight block provides a way for detailed animation of Light Sources, such as the indicator, brake, fog and main lights of a vehicle, or a light post.
      |
      | For more information, please click Help.
      settings: OpenFcn=open_system([gcb '/Actuator'],'mask')
      mask Help: eval('openHelp(209)')
      mask Display: image(imread('HeadLight.png'))
  Mazda_RX8_1_Indicator_side_left : Subsystem  Tag=actuator/IndicatorSL  Priority=0  LoadFcn=load('PreScanVisuLightActuatorData');load('PrescanRPYData');load('PrescanXYZData');load('PreScanRGBData')  mask(PreScan Sink Block: VisuActiveLight){}
      mask help:
      | The VisuActiveLight block provides a way for detailed animation of Light Sources, such as the indicator, brake, fog and main lights of a vehicle, or a light post.
      |
      | For more information, please click Help.
      settings: OpenFcn=open_system([gcb '/Actuator'],'mask')
      mask Help: eval('openHelp(209)')
      mask Display: image(imread('HeadLight.png'))
  Mazda_RX8_1_Indicator_side_right : Subsystem  Tag=actuator/IndicatorSR  Priority=0  LoadFcn=load('PreScanVisuLightActuatorData');load('PrescanRPYData');load('PrescanXYZData');load('PreScanRGBData')  mask(PreScan Sink Block: VisuActiveLight){}
      mask help:
      | The VisuActiveLight block provides a way for detailed animation of Light Sources, such as the indicator, brake, fog and main lights of a vehicle, or a light post.
      |
      | For more information, please click Help.
      settings: OpenFcn=open_system([gcb '/Actuator'],'mask')
      mask Help: eval('openHelp(209)')
      mask Display: image(imread('HeadLight.png'))
  PreScanTerminator : Subsystem  Tag=PreScanTerminator  Priority=999  LoadFcn=load PrescanTerminatorData  mask(PreScan Simulation Terminator){TimeStep=1/100}
      mask prompts: TimeStep "Upload Period [s]"
      mask help:
      | Please do not remove this block from the compilation sheet as it
      | connects the model to the PreScan environment.
      mask Help: eval('openHelp(812)')
      mask Display: image(imread('prescanlogo.ico'))
  SELF_Audi_A8_1 : Subsystem  Tag=sensor/SelfPort  Priority=30  LoadFcn=load('PreScanSelfSensorData.mat')  mask(PreScan Source Block: SELF){}
      mask help:
      | The SELF port shows (state) information of the actor itself. The outputs are position in the experiment's axis system and the GPS coordinates, and the object's absolute velocity and compass heading.
      |
      | For more information, please click Help.
      settings: OpenFcn=open_system([gcb '/Sensor'],'mask')
      mask Help: eval('openHelp(462)')
      mask Display: image(imread('GPS.png'))
  SELF_BMW_X5_1 : Subsystem  Tag=sensor/SelfPort  Priority=30  LoadFcn=load('PreScanSelfSensorData.mat')  mask(PreScan Source Block: SELF){}
      mask help:
      | The SELF port shows (state) information of the actor itself. The outputs are position in the experiment's axis system and the GPS coordinates, and the object's absolute velocity and compass heading.
      |
      | For more information, please click Help.
      settings: OpenFcn=open_system([gcb '/Sensor'],'mask')
      mask Help: eval('openHelp(462)')
      mask Display: image(imread('GPS.png'))
  SELF_Fiat_Bravo_1 : Subsystem  Tag=sensor/SelfPort  Priority=30  LoadFcn=load('PreScanSelfSensorData.mat')  mask(PreScan Source Block: SELF){}
      mask help:
      | The SELF port shows (state) information of the actor itself. The outputs are position in the experiment's axis system and the GPS coordinates, and the object's absolute velocity and compass heading.
      |
      | For more information, please click Help.
      settings: OpenFcn=open_system([gcb '/Sensor'],'mask')
      mask Help: eval('openHelp(462)')
      mask Display: image(imread('GPS.png'))
  SELF_Ford_Fiesta_1 : Subsystem  Tag=sensor/SelfPort  Priority=30  LoadFcn=load('PreScanSelfSensorData.mat')  mask(PreScan Source Block: SELF){}
      mask help:
      | The SELF port shows (state) information of the actor itself. The outputs are position in the experiment's axis system and the GPS coordinates, and the object's absolute velocity and compass heading.
      |
      | For more information, please click Help.
      settings: OpenFcn=open_system([gcb '/Sensor'],'mask')
      mask Help: eval('openHelp(462)')
      mask Display: image(imread('GPS.png'))
  SELF_Honda_Pan_European_1 : Subsystem  Tag=sensor/SelfPort  Priority=30  LoadFcn=load('PreScanSelfSensorData.mat')  mask(PreScan Source Block: SELF){}
      mask help:
      | The SELF port shows (state) information of the actor itself. The outputs are position in the experiment's axis system and the GPS coordinates, and the object's absolute velocity and compass heading.
      |
      | For more information, please click Help.
      settings: OpenFcn=open_system([gcb '/Sensor'],'mask')
      mask Help: eval('openHelp(462)')
      mask Display: image(imread('GPS.png'))
  SELF_Mazda_RX8_1 : Subsystem  Tag=sensor/SelfPort  Priority=30  LoadFcn=load('PreScanSelfSensorData.mat')  mask(PreScan Source Block: SELF){}
      mask help:
      | The SELF port shows (state) information of the actor itself. The outputs are position in the experiment's axis system and the GPS coordinates, and the object's absolute velocity and compass heading.
      |
      | For more information, please click Help.
      settings: OpenFcn=open_system([gcb '/Sensor'],'mask')
      mask Help: eval('openHelp(462)')
      mask Display: image(imread('GPS.png'))
  SELF_Sphere_1 : Subsystem  Tag=sensor/SelfPort  Priority=30  LoadFcn=load('PreScanSelfSensorData.mat')  mask(PreScan Source Block: SELF){}
      mask help:
      | The SELF port shows (state) information of the actor itself. The outputs are position in the experiment's axis system and the GPS coordinates, and the object's absolute velocity and compass heading.
      |
      | For more information, please click Help.
      settings: OpenFcn=open_system([gcb '/Sensor'],'mask')
      mask Help: eval('openHelp(462)')
      mask Display: image(imread('GPS.png'))
  SELF_Toyota_Yaris_1 : Subsystem  Tag=sensor/SelfPort  Priority=30  LoadFcn=load('PreScanSelfSensorData.mat')  mask(PreScan Source Block: SELF){}
      mask help:
      | The SELF port shows (state) information of the actor itself. The outputs are position in the experiment's axis system and the GPS coordinates, and the object's absolute velocity and compass heading.
      |
      | For more information, please click Help.
      settings: OpenFcn=open_system([gcb '/Sensor'],'mask')
      mask Help: eval('openHelp(462)')
      mask Display: image(imread('GPS.png'))
  STATE_Audi_A8_1_bus : Subsystem  Tag=actuator/StatePort  Priority=0  LoadFcn=load('PreScanStateActuatorData.mat')  mask(PreScan Sink Block: State){}
      mask help:
      | The Actor State contains a vector signal of size (9x1), containing the following signals:
      |
      | -  Position    	(x,y,z)             	[m]
      | -  Velocity    	(vx,vy,vz)         	[m/s]
      | -  Angles       	(Roll, Pitch, Yaw)	[rad]
      |
      | The Actor state is defined in the global axis system.
      | The state is superponed on the Initial position defined in the GUI.
      |
      | For more information, please click Help.
      settings: OpenFcn=open_system([gcb '/Actuator'],'mask')
      mask Help: eval('openHelp(222)')
      mask Display: image(imread('State.png'))
  STATE_BMW_X5_1_bus : Subsystem  Tag=actuator/StatePort  Priority=0  LoadFcn=load('PreScanStateActuatorData.mat')  mask(PreScan Sink Block: State){}
      mask help:
      | The Actor State contains a vector signal of size (9x1), containing the following signals:
      |
      | -  Position    	(x,y,z)             	[m]
      | -  Velocity    	(vx,vy,vz)         	[m/s]
      | -  Angles       	(Roll, Pitch, Yaw)	[rad]
      |
      | The Actor state is defined in the global axis system.
      | The state is superponed on the Initial position defined in the GUI.
      |
      | For more information, please click Help.
      settings: OpenFcn=open_system([gcb '/Actuator'],'mask')
      mask Help: eval('openHelp(222)')
      mask Display: image(imread('State.png'))
  STATE_Fiat_Bravo_1_bus : Subsystem  Tag=actuator/StatePort  Priority=0  LoadFcn=load('PreScanStateActuatorData.mat')  mask(PreScan Sink Block: State){}
      mask help:
      | The Actor State contains a vector signal of size (9x1), containing the following signals:
      |
      | -  Position    	(x,y,z)             	[m]
      | -  Velocity    	(vx,vy,vz)         	[m/s]
      | -  Angles       	(Roll, Pitch, Yaw)	[rad]
      |
      | The Actor state is defined in the global axis system.
      | The state is superponed on the Initial position defined in the GUI.
      |
      | For more information, please click Help.
      settings: OpenFcn=open_system([gcb '/Actuator'],'mask')
      mask Help: eval('openHelp(222)')
      mask Display: image(imread('State.png'))
  STATE_Ford_Fiesta_1_bus : Subsystem  Tag=actuator/StatePort  Priority=0  LoadFcn=load('PreScanStateActuatorData.mat')  mask(PreScan Sink Block: State){}
      mask help:
      | The Actor State contains a vector signal of size (9x1), containing the following signals:
      |
      | -  Position    	(x,y,z)             	[m]
      | -  Velocity    	(vx,vy,vz)         	[m/s]
      | -  Angles       	(Roll, Pitch, Yaw)	[rad]
      |
      | The Actor state is defined in the global axis system.
      | The state is superponed on the Initial position defined in the GUI.
      |
      | For more information, please click Help.
      settings: OpenFcn=open_system([gcb '/Actuator'],'mask')
      mask Help: eval('openHelp(222)')
      mask Display: image(imread('State.png'))
  STATE_Honda_Pan_European_1_bus : Subsystem  Tag=actuator/StatePort  Priority=0  LoadFcn=load('PreScanStateActuatorData.mat')  mask(PreScan Sink Block: State){}
      mask help:
      | The Actor State contains a vector signal of size (9x1), containing the following signals:
      |
      | -  Position    	(x,y,z)             	[m]
      | -  Velocity    	(vx,vy,vz)         	[m/s]
      | -  Angles       	(Roll, Pitch, Yaw)	[rad]
      |
      | The Actor state is defined in the global axis system.
      | The state is superponed on the Initial position defined in the GUI.
      |
      | For more information, please click Help.
      settings: OpenFcn=open_system([gcb '/Actuator'],'mask')
      mask Help: eval('openHelp(222)')
      mask Display: image(imread('State.png'))
  STATE_Mazda_RX8_1_bus : Subsystem  Tag=actuator/StatePort  Priority=0  LoadFcn=load('PreScanStateActuatorData.mat')  mask(PreScan Sink Block: State){}
      mask help:
      | The Actor State contains a vector signal of size (9x1), containing the following signals:
      |
      | -  Position    	(x,y,z)             	[m]
      | -  Velocity    	(vx,vy,vz)         	[m/s]
      | -  Angles       	(Roll, Pitch, Yaw)	[rad]
      |
      | The Actor state is defined in the global axis system.
      | The state is superponed on the Initial position defined in the GUI.
      |
      | For more information, please click Help.
      settings: OpenFcn=open_system([gcb '/Actuator'],'mask')
      mask Help: eval('openHelp(222)')
      mask Display: image(imread('State.png'))
  STATE_Sphere_1_bus : Subsystem  Tag=actuator/StatePort  Priority=0  LoadFcn=load('PreScanStateActuatorData.mat')  mask(PreScan Sink Block: State){}
      mask help:
      | The Actor State contains a vector signal of size (9x1), containing the following signals:
      |
      | -  Position    	(x,y,z)             	[m]
      | -  Velocity    	(vx,vy,vz)         	[m/s]
      | -  Angles       	(Roll, Pitch, Yaw)	[rad]
      |
      | The Actor state is defined in the global axis system.
      | The state is superponed on the Initial position defined in the GUI.
      |
      | For more information, please click Help.
      settings: OpenFcn=open_system([gcb '/Actuator'],'mask')
      mask Help: eval('openHelp(222)')
      mask Display: image(imread('State.png'))
  STATE_Toyota_Yaris_1_bus : Subsystem  Tag=actuator/StatePort  Priority=0  LoadFcn=load('PreScanStateActuatorData.mat')  mask(PreScan Sink Block: State){}
      mask help:
      | The Actor State contains a vector signal of size (9x1), containing the following signals:
      |
      | -  Position    	(x,y,z)             	[m]
      | -  Velocity    	(vx,vy,vz)         	[m/s]
      | -  Angles       	(Roll, Pitch, Yaw)	[rad]
      |
      | The Actor state is defined in the global axis system.
      | The state is superponed on the Initial position defined in the GUI.
      |
      | For more information, please click Help.
      settings: OpenFcn=open_system([gcb '/Actuator'],'mask')
      mask Help: eval('openHelp(222)')
      mask Display: image(imread('State.png'))
  ScenarioEngine : Subsystem  Tag=PreScanOpenScenarioBlock  Priority=10  LoadFcn=load PrescanSynchronizeData  mask(PreScan Simulation Core Block){TimeStep=1/100}
      mask prompts: TimeStep "Timestep [s]"
      mask help:
      | Please do not remove this block from the PreScan compilation sheet,
      | as it contains essential configuration parameters for a PreScan simulation.
      settings: DeleteFcn=PreScanBlockDeleteFcn;
      mask Display: image(imread('prescanlogo.ico'))
  Sphere_1 : Subsystem  Tag=WorldObjectSubSystem  InitFcn=UniqueId = '24';
      mask init:
      | imagePath=which('Sphere.jpg');
      mask Display: image(imread(imagePath));color('white');text(0, 0, ' ID=5\n')
  SteeringColumn_pivot_Audi_A8_1 : Subsystem  Tag=Actuator  Priority=0  LoadFcn=load('PrescanPoseData');load('PrescanXYZData');load('PreScanRPYData')
      mask help:
      | The VisuJoint block provides a way to adapt the location and orientation of a part of an object.
      |
      | For more information, please click Help.
      settings: OpenFcn=open_system([gcb '/Actuator'],'mask')
      mask Display: image(imread('Joint.png'))
  SteeringColumn_pivot_BMW_X5_1 : Subsystem  Tag=Actuator  Priority=0  LoadFcn=load('PrescanPoseData');load('PrescanXYZData');load('PreScanRPYData')
      mask help:
      | The VisuJoint block provides a way to adapt the location and orientation of a part of an object.
      |
      | For more information, please click Help.
      settings: OpenFcn=open_system([gcb '/Actuator'],'mask')
      mask Display: image(imread('Joint.png'))
  SteeringColumn_pivot_Fiat_Bravo_1 : Subsystem  Tag=Actuator  Priority=0  LoadFcn=load('PrescanPoseData');load('PrescanXYZData');load('PreScanRPYData')
      mask help:
      | The VisuJoint block provides a way to adapt the location and orientation of a part of an object.
      |
      | For more information, please click Help.
      settings: OpenFcn=open_system([gcb '/Actuator'],'mask')
      mask Display: image(imread('Joint.png'))
  SteeringColumn_pivot_Ford_Fiesta_1 : Subsystem  Tag=Actuator  Priority=0  LoadFcn=load('PrescanPoseData');load('PrescanXYZData');load('PreScanRPYData')
      mask help:
      | The VisuJoint block provides a way to adapt the location and orientation of a part of an object.
      |
      | For more information, please click Help.
      settings: OpenFcn=open_system([gcb '/Actuator'],'mask')
      mask Display: image(imread('Joint.png'))
  SteeringColumn_pivot_Honda_Pan_European_1 : Subsystem  Tag=Actuator  Priority=0  LoadFcn=load('PrescanPoseData');load('PrescanXYZData');load('PreScanRPYData')
      mask help:
      | The VisuJoint block provides a way to adapt the location and orientation of a part of an object.
      |
      | For more information, please click Help.
      settings: OpenFcn=open_system([gcb '/Actuator'],'mask')
      mask Display: image(imread('Joint.png'))
  SteeringColumn_pivot_Mazda_RX8_1 : Subsystem  Tag=Actuator  Priority=0  LoadFcn=load('PrescanPoseData');load('PrescanXYZData');load('PreScanRPYData')
      mask help:
      | The VisuJoint block provides a way to adapt the location and orientation of a part of an object.
      |
      | For more information, please click Help.
      settings: OpenFcn=open_system([gcb '/Actuator'],'mask')
      mask Display: image(imread('Joint.png'))
  SteeringColumn_pivot_Toyota_Yaris_1 : Subsystem  Tag=Actuator  Priority=0  LoadFcn=load('PrescanPoseData');load('PrescanXYZData');load('PreScanRPYData')
      mask help:
      | The VisuJoint block provides a way to adapt the location and orientation of a part of an object.
      |
      | For more information, please click Help.
      settings: OpenFcn=open_system([gcb '/Actuator'],'mask')
      mask Display: image(imread('Joint.png'))
  SteeringWheel_pivot_Audi_A8_1 : Subsystem  Tag=Actuator  Priority=0  LoadFcn=load('PrescanPoseData');load('PrescanXYZData');load('PreScanRPYData')
      mask help:
      | The VisuJoint block provides a way to adapt the location and orientation of a part of an object.
      |
      | For more information, please click Help.
      settings: OpenFcn=open_system([gcb '/Actuator'],'mask')
      mask Display: image(imread('Joint.png'))
  SteeringWheel_pivot_BMW_X5_1 : Subsystem  Tag=Actuator  Priority=0  LoadFcn=load('PrescanPoseData');load('PrescanXYZData');load('PreScanRPYData')
      mask help:
      | The VisuJoint block provides a way to adapt the location and orientation of a part of an object.
      |
      | For more information, please click Help.
      settings: OpenFcn=open_system([gcb '/Actuator'],'mask')
      mask Display: image(imread('Joint.png'))
  SteeringWheel_pivot_Fiat_Bravo_1 : Subsystem  Tag=Actuator  Priority=0  LoadFcn=load('PrescanPoseData');load('PrescanXYZData');load('PreScanRPYData')
      mask help:
      | The VisuJoint block provides a way to adapt the location and orientation of a part of an object.
      |
      | For more information, please click Help.
      settings: OpenFcn=open_system([gcb '/Actuator'],'mask')
      mask Display: image(imread('Joint.png'))
  SteeringWheel_pivot_Ford_Fiesta_1 : Subsystem  Tag=Actuator  Priority=0  LoadFcn=load('PrescanPoseData');load('PrescanXYZData');load('PreScanRPYData')
      mask help:
      | The VisuJoint block provides a way to adapt the location and orientation of a part of an object.
      |
      | For more information, please click Help.
      settings: OpenFcn=open_system([gcb '/Actuator'],'mask')
      mask Display: image(imread('Joint.png'))
  SteeringWheel_pivot_Mazda_RX8_1 : Subsystem  Tag=Actuator  Priority=0  LoadFcn=load('PrescanPoseData');load('PrescanXYZData');load('PreScanRPYData')
      mask help:
      | The VisuJoint block provides a way to adapt the location and orientation of a part of an object.
      |
      | For more information, please click Help.
      settings: OpenFcn=open_system([gcb '/Actuator'],'mask')
      mask Display: image(imread('Joint.png'))
  SteeringWheel_pivot_Toyota_Yaris_1 : Subsystem  Tag=Actuator  Priority=0  LoadFcn=load('PrescanPoseData');load('PrescanXYZData');load('PreScanRPYData')
      mask help:
      | The VisuJoint block provides a way to adapt the location and orientation of a part of an object.
      |
      | For more information, please click Help.
      settings: OpenFcn=open_system([gcb '/Actuator'],'mask')
      mask Display: image(imread('Joint.png'))
  Synchronizer : Subsystem  Tag=PreScanSynchronizer  Priority=20  LoadFcn=load PrescanSynchronizeData  mask(PreScan Simulation Core Block){TimeStep=1/100}
      mask prompts: TimeStep "Timestep [s]"
      mask help:
      | Please do not remove this block from the PreScan compilation sheet,
      | as it contains essential configuration parameters for a PreScan simulation.
      settings: DeleteFcn=PreScanBlockDeleteFcn;
      mask Display: image(imread('prescanlogo.ico'))
  TIS_1 : Subsystem  Tag=sensor/TIS  Priority=30  LoadFcn=load('PrescanScannerSensorData.mat');load('PrescanScannerSensorMessage.mat')  mask(PreScan Source Block: Technology Independent Sensor (TIS)){}
      mask help:
      | The Technology Independent Sensor (TIS) provides a sensor with all sensor-related influence factors (like noise, drift and accuracy) without being technology specific (like radar and lidar). The TIS detects the closest point on the geometry of an object.
      |
      | For more information, please click Help.
      settings: OpenFcn=open_system([gcb '/Sensor'],'mask')
      mask Help: eval('openHelp(449)')
      mask Display: image(imread('TIS.png'))
  TIS_2 : Subsystem  Tag=sensor/TIS  Priority=30  LoadFcn=load('PrescanScannerSensorData.mat');load('PrescanScannerSensorMessage.mat')  mask(PreScan Source Block: Technology Independent Sensor (TIS)){}
      mask help:
      | The Technology Independent Sensor (TIS) provides a sensor with all sensor-related influence factors (like noise, drift and accuracy) without being technology specific (like radar and lidar). The TIS detects the closest point on the geometry of an object.
      |
      | For more information, please click Help.
      settings: OpenFcn=open_system([gcb '/Sensor'],'mask')
      mask Help: eval('openHelp(449)')
      mask Display: image(imread('TIS.png'))
  Toyota_Yaris_1 : Subsystem  Tag=WorldObjectSubSystem  InitFcn=UniqueId = '359';
      mask init:
      | modelPath = GenericModelHelper.getGenericModelFilePath('ModelDepo','Vehicles\Toyota_Yaris\Toyota_Yaris.pgmb','3ea2b9be97d70b5ca322b210574befd9');imagePath = GenericModelHelper.getCompilationPicture(modelPath, 'Toyota_Yaris_HighPoly.png');
      mask Display: image(imread(imagePath));color('white');text(0, 0, ' ID=234\n')
  Toyota_Yaris_1_Brake_light_left : Subsystem  Tag=actuator/BrakeLightL_Pivot  Priority=0  LoadFcn=load('PreScanVisuLightActuatorData');load('PrescanRPYData');load('PrescanXYZData');load('PreScanRGBData')  mask(PreScan Sink Block: VisuActiveLight){}
      mask help:
      | The VisuActiveLight block provides a way for detailed animation of Light Sources, such as the indicator, brake, fog and main lights of a vehicle, or a light post.
      |
      | For more information, please click Help.
      settings: OpenFcn=open_system([gcb '/Actuator'],'mask')
      mask Help: eval('openHelp(209)')
      mask Display: image(imread('HeadLight.png'))
  Toyota_Yaris_1_Brake_light_right : Subsystem  Tag=actuator/BrakeLightR_Pivot  Priority=0  LoadFcn=load('PreScanVisuLightActuatorData');load('PrescanRPYData');load('PrescanXYZData');load('PreScanRGBData')  mask(PreScan Sink Block: VisuActiveLight){}
      mask help:
      | The VisuActiveLight block provides a way for detailed animation of Light Sources, such as the indicator, brake, fog and main lights of a vehicle, or a light post.
      |
      | For more information, please click Help.
      settings: OpenFcn=open_system([gcb '/Actuator'],'mask')
      mask Help: eval('openHelp(209)')
      mask Display: image(imread('HeadLight.png'))
  Toyota_Yaris_1_Indicator_front_left : Subsystem  Tag=actuator/IndicatorFL_Pivot  Priority=0  LoadFcn=load('PreScanVisuLightActuatorData');load('PrescanRPYData');load('PrescanXYZData');load('PreScanRGBData')  mask(PreScan Sink Block: VisuActiveLight){}
      mask help:
      | The VisuActiveLight block provides a way for detailed animation of Light Sources, such as the indicator, brake, fog and main lights of a vehicle, or a light post.
      |
      | For more information, please click Help.
      settings: OpenFcn=open_system([gcb '/Actuator'],'mask')
      mask Help: eval('openHelp(209)')
      mask Display: image(imread('HeadLight.png'))
  Toyota_Yaris_1_Indicator_front_right : Subsystem  Tag=actuator/IndicatorFR_Pivot  Priority=0  LoadFcn=load('PreScanVisuLightActuatorData');load('PrescanRPYData');load('PrescanXYZData');load('PreScanRGBData')  mask(PreScan Sink Block: VisuActiveLight){}
      mask help:
      | The VisuActiveLight block provides a way for detailed animation of Light Sources, such as the indicator, brake, fog and main lights of a vehicle, or a light post.
      |
      | For more information, please click Help.
      settings: OpenFcn=open_system([gcb '/Actuator'],'mask')
      mask Help: eval('openHelp(209)')
      mask Display: image(imread('HeadLight.png'))
  Toyota_Yaris_1_Indicator_rear_left : Subsystem  Tag=actuator/IndicatorRL_Pivot  Priority=0  LoadFcn=load('PreScanVisuLightActuatorData');load('PrescanRPYData');load('PrescanXYZData');load('PreScanRGBData')  mask(PreScan Sink Block: VisuActiveLight){}
      mask help:
      | The VisuActiveLight block provides a way for detailed animation of Light Sources, such as the indicator, brake, fog and main lights of a vehicle, or a light post.
      |
      | For more information, please click Help.
      settings: OpenFcn=open_system([gcb '/Actuator'],'mask')
      mask Help: eval('openHelp(209)')
      mask Display: image(imread('HeadLight.png'))
  Toyota_Yaris_1_Indicator_rear_right : Subsystem  Tag=actuator/IndicatorRR_Pivot  Priority=0  LoadFcn=load('PreScanVisuLightActuatorData');load('PrescanRPYData');load('PrescanXYZData');load('PreScanRGBData')  mask(PreScan Sink Block: VisuActiveLight){}
      mask help:
      | The VisuActiveLight block provides a way for detailed animation of Light Sources, such as the indicator, brake, fog and main lights of a vehicle, or a light post.
      |
      | For more information, please click Help.
      settings: OpenFcn=open_system([gcb '/Actuator'],'mask')
      mask Help: eval('openHelp(209)')
      mask Display: image(imread('HeadLight.png'))
  Toyota_Yaris_1_Indicator_side_left : Subsystem  Tag=actuator/IndicatorSL_Pivot  Priority=0  LoadFcn=load('PreScanVisuLightActuatorData');load('PrescanRPYData');load('PrescanXYZData');load('PreScanRGBData')  mask(PreScan Sink Block: VisuActiveLight){}
      mask help:
      | The VisuActiveLight block provides a way for detailed animation of Light Sources, such as the indicator, brake, fog and main lights of a vehicle, or a light post.
      |
      | For more information, please click Help.
      settings: OpenFcn=open_system([gcb '/Actuator'],'mask')
      mask Help: eval('openHelp(209)')
      mask Display: image(imread('HeadLight.png'))
  Toyota_Yaris_1_Indicator_side_right : Subsystem  Tag=actuator/IndicatorSR_Pivot  Priority=0  LoadFcn=load('PreScanVisuLightActuatorData');load('PrescanRPYData');load('PrescanXYZData');load('PreScanRGBData')  mask(PreScan Sink Block: VisuActiveLight){}
      mask help:
      | The VisuActiveLight block provides a way for detailed animation of Light Sources, such as the indicator, brake, fog and main lights of a vehicle, or a light post.
      |
      | For more information, please click Help.
      settings: OpenFcn=open_system([gcb '/Actuator'],'mask')
      mask Help: eval('openHelp(209)')
      mask Display: image(imread('HeadLight.png'))
  VISUMatrixSignLights_HighwayOverhang_1 : Subsystem  Tag=actuator/VisuMatrixSignLights  Priority=0  mask(PreScan Sink Block: VisuMatrixSignLights){UniqueID=109, ColorsObjectQuery=, Colors=[]}
      mask prompts: UniqueID "Parent Unique Identifier"; ColorsObjectQuery "Query for Color Object"; Colors "Matrix of colors"
      mask help:
      | The VisuMatrixSignLights block provides a way to switch the lights on the matrix sign board on or off
      |
      | For more information, please click Help.
      settings: OpenFcn=open_system([gcb '/Actuator'],'mask')
      mask Help: eval('openHelp(732)')
      mask Display: image(imread('RearLight.png'))
  VISUMatrixSignLights_HighwayOverhang_11 : Subsystem  Tag=actuator/VisuMatrixSignLights  Priority=0  mask(PreScan Sink Block: VisuMatrixSignLights){UniqueID=120, ColorsObjectQuery=, Colors=[]}
      mask prompts: UniqueID "Parent Unique Identifier"; ColorsObjectQuery "Query for Color Object"; Colors "Matrix of colors"
      mask help:
      | The VisuMatrixSignLights block provides a way to switch the lights on the matrix sign board on or off
      |
      | For more information, please click Help.
      settings: OpenFcn=open_system([gcb '/Actuator'],'mask')
      mask Help: eval('openHelp(732)')
      mask Display: image(imread('RearLight.png'))
  VISUMatrixSignLights_HighwayOverhang_12 : Subsystem  Tag=actuator/VisuMatrixSignLights  Priority=0  mask(PreScan Sink Block: VisuMatrixSignLights){UniqueID=121, ColorsObjectQuery=, Colors=[]}
      mask prompts: UniqueID "Parent Unique Identifier"; ColorsObjectQuery "Query for Color Object"; Colors "Matrix of colors"
      mask help:
      | The VisuMatrixSignLights block provides a way to switch the lights on the matrix sign board on or off
      |
      | For more information, please click Help.
      settings: OpenFcn=open_system([gcb '/Actuator'],'mask')
      mask Help: eval('openHelp(732)')
      mask Display: image(imread('RearLight.png'))
  VISUMatrixSignLights_HighwayOverhang_2 : Subsystem  Tag=actuator/VisuMatrixSignLights  Priority=0  mask(PreScan Sink Block: VisuMatrixSignLights){UniqueID=110, ColorsObjectQuery=, Colors=[]}
      mask prompts: UniqueID "Parent Unique Identifier"; ColorsObjectQuery "Query for Color Object"; Colors "Matrix of colors"
      mask help:
      | The VisuMatrixSignLights block provides a way to switch the lights on the matrix sign board on or off
      |
      | For more information, please click Help.
      settings: OpenFcn=open_system([gcb '/Actuator'],'mask')
      mask Help: eval('openHelp(732)')
      mask Display: image(imread('RearLight.png'))
  VISUMatrixSign_HighwayOverhang_1 : Subsystem  Tag=actuator/VisuMatrixSign  Priority=0  mask(PreScan Sink Block: VisuMatrixSign){UniqueID=109, ResourceList={'1' 'InformationSign\MatrixSign_GreenArrow.png' '2' 'InformationSign\sign1.jpg' '3' 'InformationSign\sign2.jpg' '4' 'InformationSign\sign3.jpg' '5' 'InformationSign\sign10.png' '7' 'InformationSign\SEARCH_Logo.png' '8' 'InformationSign\sharp_edges.jpg' '9' 'InformationSign\road_surprises.jpg' '10' 'InformationSign\sign5.JPG' '11' 'InformationSign\tacos.jpg' '12' 'InformationSign\dont_even_think.jpg' '13' 'InformationSign\cthulhuwarn.jpg' '14' 'InformationSign\sign7.JPG' '15' 'InformationSign\sign32.jpg' '16' 'InformationSign\NoParking.jpg' '17' 'InformationSign\TheFuture.jpg' '18' 'InformationSign\sign4.jpg' '19' 'InformationSign\sign31.jpg' '20' 'InformationSign\Empty.jpeg' }, PivotName=}
      mask prompts: UniqueID "Parent Unique Identifier (auto-generated)"; ResourceList "Resource List (auto-generated)"; PivotName "Name of pivot (auto-generated)"
      mask help:
      | The VisuMatrixSign block provides a way to adapt the texture of the plates connected to an overhang, based on Resource IDs of the texture files.
      |
      | For more information, please click Help.
      settings: OpenFcn=open_system([gcb '/Actuator'],'mask')
      mask Help: eval('openHelp(733)')
      mask Display: image(imread('HighwaySpeedMatrix.png'))
  VISUMatrixSign_HighwayOverhang_10 : Subsystem  Tag=actuator/VisuMatrixSign  Priority=0  mask(PreScan Sink Block: VisuMatrixSign){UniqueID=119, ResourceList={'1' 'InformationSign\MatrixSign_GreenArrow.png' '2' 'InformationSign\sign1.jpg' '3' 'InformationSign\sign2.jpg' '4' 'InformationSign\sign3.jpg' '5' 'InformationSign\sign10.png' '7' 'InformationSign\SEARCH_Logo.png' '8' 'InformationSign\sharp_edges.jpg' '9' 'InformationSign\road_surprises.jpg' '10' 'InformationSign\sign5.JPG' '11' 'InformationSign\tacos.jpg' '12' 'InformationSign\dont_even_think.jpg' '13' 'InformationSign\cthulhuwarn.jpg' '14' 'InformationSign\sign7.JPG' '15' 'InformationSign\sign32.jpg' '16' 'InformationSign\NoParking.jpg' '17' 'InformationSign\TheFuture.jpg' '18' 'InformationSign\sign4.jpg' '19' 'InformationSign\sign31.jpg' '20' 'InformationSign\Empty.jpeg' }, PivotName=}
      mask prompts: UniqueID "Parent Unique Identifier (auto-generated)"; ResourceList "Resource List (auto-generated)"; PivotName "Name of pivot (auto-generated)"
      mask help:
      | The VisuMatrixSign block provides a way to adapt the texture of the plates connected to an overhang, based on Resource IDs of the texture files.
      |
      | For more information, please click Help.
      settings: OpenFcn=open_system([gcb '/Actuator'],'mask')
      mask Help: eval('openHelp(733)')
      mask Display: image(imread('HighwaySpeedMatrix.png'))
  VISUMatrixSign_HighwayOverhang_11 : Subsystem  Tag=actuator/VisuMatrixSign  Priority=0  mask(PreScan Sink Block: VisuMatrixSign){UniqueID=120, ResourceList={'1' 'InformationSign\MatrixSign_GreenArrow.png' '2' 'InformationSign\sign1.jpg' '3' 'InformationSign\sign2.jpg' '4' 'InformationSign\sign3.jpg' '5' 'InformationSign\sign10.png' '7' 'InformationSign\SEARCH_Logo.png' '8' 'InformationSign\sharp_edges.jpg' '9' 'InformationSign\road_surprises.jpg' '10' 'InformationSign\sign5.JPG' '11' 'InformationSign\tacos.jpg' '12' 'InformationSign\dont_even_think.jpg' '13' 'InformationSign\cthulhuwarn.jpg' '14' 'InformationSign\sign7.JPG' '15' 'InformationSign\sign32.jpg' '16' 'InformationSign\NoParking.jpg' '17' 'InformationSign\TheFuture.jpg' '18' 'InformationSign\sign4.jpg' '19' 'InformationSign\sign31.jpg' '20' 'InformationSign\Empty.jpeg' }, PivotName=}
      mask prompts: UniqueID "Parent Unique Identifier (auto-generated)"; ResourceList "Resource List (auto-generated)"; PivotName "Name of pivot (auto-generated)"
      mask help:
      | The VisuMatrixSign block provides a way to adapt the texture of the plates connected to an overhang, based on Resource IDs of the texture files.
      |
      | For more information, please click Help.
      settings: OpenFcn=open_system([gcb '/Actuator'],'mask')
      mask Help: eval('openHelp(733)')
      mask Display: image(imread('HighwaySpeedMatrix.png'))
  VISUMatrixSign_HighwayOverhang_12 : Subsystem  Tag=actuator/VisuMatrixSign  Priority=0  mask(PreScan Sink Block: VisuMatrixSign){UniqueID=121, ResourceList={'1' 'InformationSign\MatrixSign_GreenArrow.png' '2' 'InformationSign\sign1.jpg' '3' 'InformationSign\sign2.jpg' '4' 'InformationSign\sign3.jpg' '5' 'InformationSign\sign10.png' '7' 'InformationSign\SEARCH_Logo.png' '8' 'InformationSign\sharp_edges.jpg' '9' 'InformationSign\road_surprises.jpg' '10' 'InformationSign\sign5.JPG' '11' 'InformationSign\tacos.jpg' '12' 'InformationSign\dont_even_think.jpg' '13' 'InformationSign\cthulhuwarn.jpg' '14' 'InformationSign\sign7.JPG' '15' 'InformationSign\sign32.jpg' '16' 'InformationSign\NoParking.jpg' '17' 'InformationSign\TheFuture.jpg' '18' 'InformationSign\sign4.jpg' '19' 'InformationSign\sign31.jpg' '20' 'InformationSign\Empty.jpeg' }, PivotName=}
      mask prompts: UniqueID "Parent Unique Identifier (auto-generated)"; ResourceList "Resource List (auto-generated)"; PivotName "Name of pivot (auto-generated)"
      mask help:
      | The VisuMatrixSign block provides a way to adapt the texture of the plates connected to an overhang, based on Resource IDs of the texture files.
      |
      | For more information, please click Help.
      settings: OpenFcn=open_system([gcb '/Actuator'],'mask')
      mask Help: eval('openHelp(733)')
      mask Display: image(imread('HighwaySpeedMatrix.png'))
  VISUMatrixSign_HighwayOverhang_2 : Subsystem  Tag=actuator/VisuMatrixSign  Priority=0  mask(PreScan Sink Block: VisuMatrixSign){UniqueID=110, ResourceList={'1' 'InformationSign\MatrixSign_GreenArrow.png' '2' 'InformationSign\sign1.jpg' '3' 'InformationSign\sign2.jpg' '4' 'InformationSign\sign3.jpg' '5' 'InformationSign\sign10.png' '7' 'InformationSign\SEARCH_Logo.png' '8' 'InformationSign\sharp_edges.jpg' '9' 'InformationSign\road_surprises.jpg' '10' 'InformationSign\sign5.JPG' '11' 'InformationSign\tacos.jpg' '12' 'InformationSign\dont_even_think.jpg' '13' 'InformationSign\cthulhuwarn.jpg' '14' 'InformationSign\sign7.JPG' '15' 'InformationSign\sign32.jpg' '16' 'InformationSign\NoParking.jpg' '17' 'InformationSign\TheFuture.jpg' '18' 'InformationSign\sign4.jpg' '19' 'InformationSign\sign31.jpg' '20' 'InformationSign\Empty.jpeg' }, PivotName=}
      mask prompts: UniqueID "Parent Unique Identifier (auto-generated)"; ResourceList "Resource List (auto-generated)"; PivotName "Name of pivot (auto-generated)"
      mask help:
      | The VisuMatrixSign block provides a way to adapt the texture of the plates connected to an overhang, based on Resource IDs of the texture files.
      |
      | For more information, please click Help.
      settings: OpenFcn=open_system([gcb '/Actuator'],'mask')
      mask Help: eval('openHelp(733)')
      mask Display: image(imread('HighwaySpeedMatrix.png'))
  VISUMatrixSign_HighwayOverhang_3 : Subsystem  Tag=actuator/VisuMatrixSign  Priority=0  mask(PreScan Sink Block: VisuMatrixSign){UniqueID=112, ResourceList={'1' 'InformationSign\MatrixSign_GreenArrow.png' '2' 'InformationSign\sign1.jpg' '3' 'InformationSign\sign2.jpg' '4' 'InformationSign\sign3.jpg' '5' 'InformationSign\sign10.png' '7' 'InformationSign\SEARCH_Logo.png' '8' 'InformationSign\sharp_edges.jpg' '9' 'InformationSign\road_surprises.jpg' '10' 'InformationSign\sign5.JPG' '11' 'InformationSign\tacos.jpg' '12' 'InformationSign\dont_even_think.jpg' '13' 'InformationSign\cthulhuwarn.jpg' '14' 'InformationSign\sign7.JPG' '15' 'InformationSign\sign32.jpg' '16' 'InformationSign\NoParking.jpg' '17' 'InformationSign\TheFuture.jpg' '18' 'InformationSign\sign4.jpg' '19' 'InformationSign\sign31.jpg' '20' 'InformationSign\Empty.jpeg' }, PivotName=}
      mask prompts: UniqueID "Parent Unique Identifier (auto-generated)"; ResourceList "Resource List (auto-generated)"; PivotName "Name of pivot (auto-generated)"
      mask help:
      | The VisuMatrixSign block provides a way to adapt the texture of the plates connected to an overhang, based on Resource IDs of the texture files.
      |
      | For more information, please click Help.
      settings: OpenFcn=open_system([gcb '/Actuator'],'mask')
      mask Help: eval('openHelp(733)')
      mask Display: image(imread('HighwaySpeedMatrix.png'))
  VISUMatrixSign_HighwayOverhang_4 : Subsystem  Tag=actuator/VisuMatrixSign  Priority=0  mask(PreScan Sink Block: VisuMatrixSign){UniqueID=113, ResourceList={'1' 'InformationSign\MatrixSign_GreenArrow.png' '2' 'InformationSign\sign1.jpg' '3' 'InformationSign\sign2.jpg' '4' 'InformationSign\sign3.jpg' '5' 'InformationSign\sign10.png' '7' 'InformationSign\SEARCH_Logo.png' '8' 'InformationSign\sharp_edges.jpg' '9' 'InformationSign\road_surprises.jpg' '10' 'InformationSign\sign5.JPG' '11' 'InformationSign\tacos.jpg' '12' 'InformationSign\dont_even_think.jpg' '13' 'InformationSign\cthulhuwarn.jpg' '14' 'InformationSign\sign7.JPG' '15' 'InformationSign\sign32.jpg' '16' 'InformationSign\NoParking.jpg' '17' 'InformationSign\TheFuture.jpg' '18' 'InformationSign\sign4.jpg' '19' 'InformationSign\sign31.jpg' '20' 'InformationSign\Empty.jpeg' }, PivotName=}
      mask prompts: UniqueID "Parent Unique Identifier (auto-generated)"; ResourceList "Resource List (auto-generated)"; PivotName "Name of pivot (auto-generated)"
      mask help:
      | The VisuMatrixSign block provides a way to adapt the texture of the plates connected to an overhang, based on Resource IDs of the texture files.
      |
      | For more information, please click Help.
      settings: OpenFcn=open_system([gcb '/Actuator'],'mask')
      mask Help: eval('openHelp(733)')
      mask Display: image(imread('HighwaySpeedMatrix.png'))
  VISUMatrixSign_HighwayOverhang_5 : Subsystem  Tag=actuator/VisuMatrixSign  Priority=0  mask(PreScan Sink Block: VisuMatrixSign){UniqueID=114, ResourceList={'1' 'InformationSign\MatrixSign_GreenArrow.png' '2' 'InformationSign\sign1.jpg' '3' 'InformationSign\sign2.jpg' '4' 'InformationSign\sign3.jpg' '5' 'InformationSign\sign10.png' '7' 'InformationSign\SEARCH_Logo.png' '8' 'InformationSign\sharp_edges.jpg' '9' 'InformationSign\road_surprises.jpg' '10' 'InformationSign\sign5.JPG' '11' 'InformationSign\tacos.jpg' '12' 'InformationSign\dont_even_think.jpg' '13' 'InformationSign\cthulhuwarn.jpg' '14' 'InformationSign\sign7.JPG' '15' 'InformationSign\sign32.jpg' '16' 'InformationSign\NoParking.jpg' '17' 'InformationSign\TheFuture.jpg' '18' 'InformationSign\sign4.jpg' '19' 'InformationSign\sign31.jpg' '20' 'InformationSign\Empty.jpeg' }, PivotName=}
      mask prompts: UniqueID "Parent Unique Identifier (auto-generated)"; ResourceList "Resource List (auto-generated)"; PivotName "Name of pivot (auto-generated)"
      mask help:
      | The VisuMatrixSign block provides a way to adapt the texture of the plates connected to an overhang, based on Resource IDs of the texture files.
      |
      | For more information, please click Help.
      settings: OpenFcn=open_system([gcb '/Actuator'],'mask')
      mask Help: eval('openHelp(733)')
      mask Display: image(imread('HighwaySpeedMatrix.png'))
  VISUMatrixSign_HighwayOverhang_6 : Subsystem  Tag=actuator/VisuMatrixSign  Priority=0  mask(PreScan Sink Block: VisuMatrixSign){UniqueID=115, ResourceList={'1' 'InformationSign\MatrixSign_GreenArrow.png' '2' 'InformationSign\sign1.jpg' '3' 'InformationSign\sign2.jpg' '4' 'InformationSign\sign3.jpg' '5' 'InformationSign\sign10.png' '7' 'InformationSign\SEARCH_Logo.png' '8' 'InformationSign\sharp_edges.jpg' '9' 'InformationSign\road_surprises.jpg' '10' 'InformationSign\sign5.JPG' '11' 'InformationSign\tacos.jpg' '12' 'InformationSign\dont_even_think.jpg' '13' 'InformationSign\cthulhuwarn.jpg' '14' 'InformationSign\sign7.JPG' '15' 'InformationSign\sign32.jpg' '16' 'InformationSign\NoParking.jpg' '17' 'InformationSign\TheFuture.jpg' '18' 'InformationSign\sign4.jpg' '19' 'InformationSign\sign31.jpg' '20' 'InformationSign\Empty.jpeg' }, PivotName=}
      mask prompts: UniqueID "Parent Unique Identifier (auto-generated)"; ResourceList "Resource List (auto-generated)"; PivotName "Name of pivot (auto-generated)"
      mask help:
      | The VisuMatrixSign block provides a way to adapt the texture of the plates connected to an overhang, based on Resource IDs of the texture files.
      |
      | For more information, please click Help.
      settings: OpenFcn=open_system([gcb '/Actuator'],'mask')
      mask Help: eval('openHelp(733)')
      mask Display: image(imread('HighwaySpeedMatrix.png'))
  VISUMatrixSign_HighwayOverhang_7 : Subsystem  Tag=actuator/VisuMatrixSign  Priority=0  mask(PreScan Sink Block: VisuMatrixSign){UniqueID=116, ResourceList={'1' 'InformationSign\MatrixSign_GreenArrow.png' '2' 'InformationSign\sign1.jpg' '3' 'InformationSign\sign2.jpg' '4' 'InformationSign\sign3.jpg' '5' 'InformationSign\sign10.png' '7' 'InformationSign\SEARCH_Logo.png' '8' 'InformationSign\sharp_edges.jpg' '9' 'InformationSign\road_surprises.jpg' '10' 'InformationSign\sign5.JPG' '11' 'InformationSign\tacos.jpg' '12' 'InformationSign\dont_even_think.jpg' '13' 'InformationSign\cthulhuwarn.jpg' '14' 'InformationSign\sign7.JPG' '15' 'InformationSign\sign32.jpg' '16' 'InformationSign\NoParking.jpg' '17' 'InformationSign\TheFuture.jpg' '18' 'InformationSign\sign4.jpg' '19' 'InformationSign\sign31.jpg' '20' 'InformationSign\Empty.jpeg' }, PivotName=}
      mask prompts: UniqueID "Parent Unique Identifier (auto-generated)"; ResourceList "Resource List (auto-generated)"; PivotName "Name of pivot (auto-generated)"
      mask help:
      | The VisuMatrixSign block provides a way to adapt the texture of the plates connected to an overhang, based on Resource IDs of the texture files.
      |
      | For more information, please click Help.
      settings: OpenFcn=open_system([gcb '/Actuator'],'mask')
      mask Help: eval('openHelp(733)')
      mask Display: image(imread('HighwaySpeedMatrix.png'))
  VISUMatrixSign_HighwayOverhang_8 : Subsystem  Tag=actuator/VisuMatrixSign  Priority=0  mask(PreScan Sink Block: VisuMatrixSign){UniqueID=117, ResourceList={'1' 'InformationSign\MatrixSign_GreenArrow.png' '2' 'InformationSign\sign1.jpg' '3' 'InformationSign\sign2.jpg' '4' 'InformationSign\sign3.jpg' '5' 'InformationSign\sign10.png' '7' 'InformationSign\SEARCH_Logo.png' '8' 'InformationSign\sharp_edges.jpg' '9' 'InformationSign\road_surprises.jpg' '10' 'InformationSign\sign5.JPG' '11' 'InformationSign\tacos.jpg' '12' 'InformationSign\dont_even_think.jpg' '13' 'InformationSign\cthulhuwarn.jpg' '14' 'InformationSign\sign7.JPG' '15' 'InformationSign\sign32.jpg' '16' 'InformationSign\NoParking.jpg' '17' 'InformationSign\TheFuture.jpg' '18' 'InformationSign\sign4.jpg' '19' 'InformationSign\sign31.jpg' '20' 'InformationSign\Empty.jpeg' }, PivotName=}
      mask prompts: UniqueID "Parent Unique Identifier (auto-generated)"; ResourceList "Resource List (auto-generated)"; PivotName "Name of pivot (auto-generated)"
      mask help:
      | The VisuMatrixSign block provides a way to adapt the texture of the plates connected to an overhang, based on Resource IDs of the texture files.
      |
      | For more information, please click Help.
      settings: OpenFcn=open_system([gcb '/Actuator'],'mask')
      mask Help: eval('openHelp(733)')
      mask Display: image(imread('HighwaySpeedMatrix.png'))
  VISUMatrixSign_HighwayOverhang_9 : Subsystem  Tag=actuator/VisuMatrixSign  Priority=0  mask(PreScan Sink Block: VisuMatrixSign){UniqueID=118, ResourceList={'1' 'InformationSign\MatrixSign_GreenArrow.png' '2' 'InformationSign\sign1.jpg' '3' 'InformationSign\sign2.jpg' '4' 'InformationSign\sign3.jpg' '5' 'InformationSign\sign10.png' '7' 'InformationSign\SEARCH_Logo.png' '8' 'InformationSign\sharp_edges.jpg' '9' 'InformationSign\road_surprises.jpg' '10' 'InformationSign\sign5.JPG' '11' 'InformationSign\tacos.jpg' '12' 'InformationSign\dont_even_think.jpg' '13' 'InformationSign\cthulhuwarn.jpg' '14' 'InformationSign\sign7.JPG' '15' 'InformationSign\sign32.jpg' '16' 'InformationSign\NoParking.jpg' '17' 'InformationSign\TheFuture.jpg' '18' 'InformationSign\sign4.jpg' '19' 'InformationSign\sign31.jpg' '20' 'InformationSign\Empty.jpeg' }, PivotName=}
      mask prompts: UniqueID "Parent Unique Identifier (auto-generated)"; ResourceList "Resource List (auto-generated)"; PivotName "Name of pivot (auto-generated)"
      mask help:
      | The VisuMatrixSign block provides a way to adapt the texture of the plates connected to an overhang, based on Resource IDs of the texture files.
      |
      | For more information, please click Help.
      settings: OpenFcn=open_system([gcb '/Actuator'],'mask')
      mask Help: eval('openHelp(733)')
      mask Display: image(imread('HighwaySpeedMatrix.png'))
  Wheel0_Honda_Pan_European_1 : Subsystem  Tag=Actuator  Priority=0  LoadFcn=load('PrescanPoseData');load('PrescanXYZData');load('PreScanRPYData')
      mask help:
      | The VisuJoint block provides a way to adapt the location and orientation of a part of an object.
      |
      | For more information, please click Help.
      settings: OpenFcn=open_system([gcb '/Actuator'],'mask')
      mask Display: image(imread('Joint.png'))
  Wheel0_Suspension_Honda_Pan_European_1 : Subsystem  Tag=Actuator  Priority=0  LoadFcn=load('PrescanPoseData');load('PrescanXYZData');load('PreScanRPYData')
      mask help:
      | The VisuJoint block provides a way to adapt the location and orientation of a part of an object.
      |
      | For more information, please click Help.
      settings: OpenFcn=open_system([gcb '/Actuator'],'mask')
      mask Display: image(imread('Joint.png'))
  Wheel1_Honda_Pan_European_1 : Subsystem  Tag=Actuator  Priority=0  LoadFcn=load('PrescanPoseData');load('PrescanXYZData');load('PreScanRPYData')
      mask help:
      | The VisuJoint block provides a way to adapt the location and orientation of a part of an object.
      |
      | For more information, please click Help.
      settings: OpenFcn=open_system([gcb '/Actuator'],'mask')
      mask Display: image(imread('Joint.png'))
  Wheel1_Suspension_Honda_Pan_European_1 : Subsystem  Tag=Actuator  Priority=0  LoadFcn=load('PrescanPoseData');load('PrescanXYZData');load('PreScanRPYData')
      mask help:
      | The VisuJoint block provides a way to adapt the location and orientation of a part of an object.
      |
      | For more information, please click Help.
      settings: OpenFcn=open_system([gcb '/Actuator'],'mask')
      mask Display: image(imread('Joint.png'))
  WheelL0_Audi_A8_1 : Subsystem  Tag=Actuator  Priority=0  LoadFcn=load('PrescanPoseData');load('PrescanXYZData');load('PreScanRPYData')
      mask help:
      | The VisuJoint block provides a way to adapt the location and orientation of a part of an object.
      |
      | For more information, please click Help.
      settings: OpenFcn=open_system([gcb '/Actuator'],'mask')
      mask Display: image(imread('Joint.png'))
  WheelL0_BMW_X5_1 : Subsystem  Tag=Actuator  Priority=0  LoadFcn=load('PrescanPoseData');load('PrescanXYZData');load('PreScanRPYData')
      mask help:
      | The VisuJoint block provides a way to adapt the location and orientation of a part of an object.
      |
      | For more information, please click Help.
      settings: OpenFcn=open_system([gcb '/Actuator'],'mask')
      mask Display: image(imread('Joint.png'))
  WheelL0_Fiat_Bravo_1 : Subsystem  Tag=Actuator  Priority=0  LoadFcn=load('PrescanPoseData');load('PrescanXYZData');load('PreScanRPYData')
      mask help:
      | The VisuJoint block provides a way to adapt the location and orientation of a part of an object.
      |
      | For more information, please click Help.
      settings: OpenFcn=open_system([gcb '/Actuator'],'mask')
      mask Display: image(imread('Joint.png'))
  WheelL0_Ford_Fiesta_1 : Subsystem  Tag=Actuator  Priority=0  LoadFcn=load('PrescanPoseData');load('PrescanXYZData');load('PreScanRPYData')
      mask help:
      | The VisuJoint block provides a way to adapt the location and orientation of a part of an object.
      |
      | For more information, please click Help.
      settings: OpenFcn=open_system([gcb '/Actuator'],'mask')
      mask Display: image(imread('Joint.png'))
  WheelL0_Mazda_RX8_1 : Subsystem  Tag=Actuator  Priority=0  LoadFcn=load('PrescanPoseData');load('PrescanXYZData');load('PreScanRPYData')
      mask help:
      | The VisuJoint block provides a way to adapt the location and orientation of a part of an object.
      |
      | For more information, please click Help.
      settings: OpenFcn=open_system([gcb '/Actuator'],'mask')
      mask Display: image(imread('Joint.png'))
  WheelL0_Toyota_Yaris_1 : Subsystem  Tag=Actuator  Priority=0  LoadFcn=load('PrescanPoseData');load('PrescanXYZData');load('PreScanRPYData')
      mask help:
      | The VisuJoint block provides a way to adapt the location and orientation of a part of an object.
      |
      | For more information, please click Help.
      settings: OpenFcn=open_system([gcb '/Actuator'],'mask')
      mask Display: image(imread('Joint.png'))
  WheelL1_Audi_A8_1 : Subsystem  Tag=Actuator  Priority=0  LoadFcn=load('PrescanPoseData');load('PrescanXYZData');load('PreScanRPYData')
      mask help:
      | The VisuJoint block provides a way to adapt the location and orientation of a part of an object.
      |
      | For more information, please click Help.
      settings: OpenFcn=open_system([gcb '/Actuator'],'mask')
      mask Display: image(imread('Joint.png'))
  WheelL1_BMW_X5_1 : Subsystem  Tag=Actuator  Priority=0  LoadFcn=load('PrescanPoseData');load('PrescanXYZData');load('PreScanRPYData')
      mask help:
      | The VisuJoint block provides a way to adapt the location and orientation of a part of an object.
      |
      | For more information, please click Help.
      settings: OpenFcn=open_system([gcb '/Actuator'],'mask')
      mask Display: image(imread('Joint.png'))
  WheelL1_Fiat_Bravo_1 : Subsystem  Tag=Actuator  Priority=0  LoadFcn=load('PrescanPoseData');load('PrescanXYZData');load('PreScanRPYData')
      mask help:
      | The VisuJoint block provides a way to adapt the location and orientation of a part of an object.
      |
      | For more information, please click Help.
      settings: OpenFcn=open_system([gcb '/Actuator'],'mask')
      mask Display: image(imread('Joint.png'))
  WheelL1_Ford_Fiesta_1 : Subsystem  Tag=Actuator  Priority=0  LoadFcn=load('PrescanPoseData');load('PrescanXYZData');load('PreScanRPYData')
      mask help:
      | The VisuJoint block provides a way to adapt the location and orientation of a part of an object.
      |
      | For more information, please click Help.
      settings: OpenFcn=open_system([gcb '/Actuator'],'mask')
      mask Display: image(imread('Joint.png'))
  WheelL1_Mazda_RX8_1 : Subsystem  Tag=Actuator  Priority=0  LoadFcn=load('PrescanPoseData');load('PrescanXYZData');load('PreScanRPYData')
      mask help:
      | The VisuJoint block provides a way to adapt the location and orientation of a part of an object.
      |
      | For more information, please click Help.
      settings: OpenFcn=open_system([gcb '/Actuator'],'mask')
      mask Display: image(imread('Joint.png'))
  WheelL1_Toyota_Yaris_1 : Subsystem  Tag=Actuator  Priority=0  LoadFcn=load('PrescanPoseData');load('PrescanXYZData');load('PreScanRPYData')
      mask help:
      | The VisuJoint block provides a way to adapt the location and orientation of a part of an object.
      |
      | For more information, please click Help.
      settings: OpenFcn=open_system([gcb '/Actuator'],'mask')
      mask Display: image(imread('Joint.png'))
  WheelR0_Audi_A8_1 : Subsystem  Tag=Actuator  Priority=0  LoadFcn=load('PrescanPoseData');load('PrescanXYZData');load('PreScanRPYData')
      mask help:
      | The VisuJoint block provides a way to adapt the location and orientation of a part of an object.
      |
      | For more information, please click Help.
      settings: OpenFcn=open_system([gcb '/Actuator'],'mask')
      mask Display: image(imread('Joint.png'))
  WheelR0_BMW_X5_1 : Subsystem  Tag=Actuator  Priority=0  LoadFcn=load('PrescanPoseData');load('PrescanXYZData');load('PreScanRPYData')
      mask help:
      | The VisuJoint block provides a way to adapt the location and orientation of a part of an object.
      |
      | For more information, please click Help.
      settings: OpenFcn=open_system([gcb '/Actuator'],'mask')
      mask Display: image(imread('Joint.png'))
  WheelR0_Fiat_Bravo_1 : Subsystem  Tag=Actuator  Priority=0  LoadFcn=load('PrescanPoseData');load('PrescanXYZData');load('PreScanRPYData')
      mask help:
      | The VisuJoint block provides a way to adapt the location and orientation of a part of an object.
      |
      | For more information, please click Help.
      settings: OpenFcn=open_system([gcb '/Actuator'],'mask')
      mask Display: image(imread('Joint.png'))
  WheelR0_Ford_Fiesta_1 : Subsystem  Tag=Actuator  Priority=0  LoadFcn=load('PrescanPoseData');load('PrescanXYZData');load('PreScanRPYData')
      mask help:
      | The VisuJoint block provides a way to adapt the location and orientation of a part of an object.
      |
      | For more information, please click Help.
      settings: OpenFcn=open_system([gcb '/Actuator'],'mask')
      mask Display: image(imread('Joint.png'))
  WheelR0_Mazda_RX8_1 : Subsystem  Tag=Actuator  Priority=0  LoadFcn=load('PrescanPoseData');load('PrescanXYZData');load('PreScanRPYData')
      mask help:
      | The VisuJoint block provides a way to adapt the location and orientation of a part of an object.
      |
      | For more information, please click Help.
      settings: OpenFcn=open_system([gcb '/Actuator'],'mask')
      mask Display: image(imread('Joint.png'))
  WheelR0_Toyota_Yaris_1 : Subsystem  Tag=Actuator  Priority=0  LoadFcn=load('PrescanPoseData');load('PrescanXYZData');load('PreScanRPYData')
      mask help:
      | The VisuJoint block provides a way to adapt the location and orientation of a part of an object.
      |
      | For more information, please click Help.
      settings: OpenFcn=open_system([gcb '/Actuator'],'mask')
      mask Display: image(imread('Joint.png'))
  WheelR1_Audi_A8_1 : Subsystem  Tag=Actuator  Priority=0  LoadFcn=load('PrescanPoseData');load('PrescanXYZData');load('PreScanRPYData')
      mask help:
      | The VisuJoint block provides a way to adapt the location and orientation of a part of an object.
      |
      | For more information, please click Help.
      settings: OpenFcn=open_system([gcb '/Actuator'],'mask')
      mask Display: image(imread('Joint.png'))
  WheelR1_BMW_X5_1 : Subsystem  Tag=Actuator  Priority=0  LoadFcn=load('PrescanPoseData');load('PrescanXYZData');load('PreScanRPYData')
      mask help:
      | The VisuJoint block provides a way to adapt the location and orientation of a part of an object.
      |
      | For more information, please click Help.
      settings: OpenFcn=open_system([gcb '/Actuator'],'mask')
      mask Display: image(imread('Joint.png'))
  WheelR1_Fiat_Bravo_1 : Subsystem  Tag=Actuator  Priority=0  LoadFcn=load('PrescanPoseData');load('PrescanXYZData');load('PreScanRPYData')
      mask help:
      | The VisuJoint block provides a way to adapt the location and orientation of a part of an object.
      |
      | For more information, please click Help.
      settings: OpenFcn=open_system([gcb '/Actuator'],'mask')
      mask Display: image(imread('Joint.png'))
  WheelR1_Ford_Fiesta_1 : Subsystem  Tag=Actuator  Priority=0  LoadFcn=load('PrescanPoseData');load('PrescanXYZData');load('PreScanRPYData')
      mask help:
      | The VisuJoint block provides a way to adapt the location and orientation of a part of an object.
      |
      | For more information, please click Help.
      settings: OpenFcn=open_system([gcb '/Actuator'],'mask')
      mask Display: image(imread('Joint.png'))
  WheelR1_Mazda_RX8_1 : Subsystem  Tag=Actuator  Priority=0  LoadFcn=load('PrescanPoseData');load('PrescanXYZData');load('PreScanRPYData')
      mask help:
      | The VisuJoint block provides a way to adapt the location and orientation of a part of an object.
      |
      | For more information, please click Help.
      settings: OpenFcn=open_system([gcb '/Actuator'],'mask')
      mask Display: image(imread('Joint.png'))
  WheelR1_Toyota_Yaris_1 : Subsystem  Tag=Actuator  Priority=0  LoadFcn=load('PrescanPoseData');load('PrescanXYZData');load('PreScanRPYData')
      mask help:
      | The VisuJoint block provides a way to adapt the location and orientation of a part of an object.
      |
      | For more information, please click Help.
      settings: OpenFcn=open_system([gcb '/Actuator'],'mask')
      mask Display: image(imread('Joint.png'))
  wires:
  Audi_A8_1/1(STATE_Audi_A8_1_bus) -> STATE_Audi_A8_1_bus/1(STATE_Audi_A8_1_bus)
  SELF_Audi_A8_1/1(SELF_Audi_A8_1) -> Audi_A8_1/1(SELF_Audi_A8_1)
  TIS_1/1(TIS_1) -> Audi_A8_1/2(TIS_1)
  TIS_2/1(TIS_2) -> Audi_A8_1/3(TIS_2)
  Audi_A8_1/2(WheelL0_Audi_A8_1) -> WheelL0_Audi_A8_1/1(WheelL0_Audi_A8_1)
  Audi_A8_1/3(WheelL1_Audi_A8_1) -> WheelL1_Audi_A8_1/1(WheelL1_Audi_A8_1)
  Audi_A8_1/4(WheelR0_Audi_A8_1) -> WheelR0_Audi_A8_1/1(WheelR0_Audi_A8_1)
  Audi_A8_1/5(WheelR1_Audi_A8_1) -> WheelR1_Audi_A8_1/1(WheelR1_Audi_A8_1)
  Audi_A8_1/6(SteeringWheel_pivot_Audi_A8_1) -> SteeringWheel_pivot_Audi_A8_1/1(SteeringWheel_pivot_Audi_A8_1)
  Audi_A8_1/7(SteeringColumn_pivot_Audi_A8_1) -> SteeringColumn_pivot_Audi_A8_1/1(SteeringColumn_pivot_Audi_A8_1)
  Audi_A8_1/8(Audi_A8_1_Brake_light_left) -> Audi_A8_1_Brake_light_left/1(Audi_A8_1_Brake_light_left)
  Audi_A8_1/9(Audi_A8_1_Brake_light_right) -> Audi_A8_1_Brake_light_right/1(Audi_A8_1_Brake_light_right)
  Audi_A8_1/10(Audi_A8_1_Indicator_front_left) -> Audi_A8_1_Indicator_front_left/1(Audi_A8_1_Indicator_front_left)
  Audi_A8_1/11(Audi_A8_1_Indicator_rear_left) -> Audi_A8_1_Indicator_rear_left/1(Audi_A8_1_Indicator_rear_left)
  Audi_A8_1/12(Audi_A8_1_Indicator_front_right) -> Audi_A8_1_Indicator_front_right/1(Audi_A8_1_Indicator_front_right)
  Audi_A8_1/13(Audi_A8_1_Indicator_rear_right) -> Audi_A8_1_Indicator_rear_right/1(Audi_A8_1_Indicator_rear_right)
  BMW_X5_1/1(STATE_BMW_X5_1_bus) -> STATE_BMW_X5_1_bus/1(STATE_BMW_X5_1_bus)
  SELF_BMW_X5_1/1(SELF_BMW_X5_1) -> BMW_X5_1/1(SELF_BMW_X5_1)
  BMW_X5_1/2(WheelL0_BMW_X5_1) -> WheelL0_BMW_X5_1/1(WheelL0_BMW_X5_1)
  BMW_X5_1/3(WheelR0_BMW_X5_1) -> WheelR0_BMW_X5_1/1(WheelR0_BMW_X5_1)
  BMW_X5_1/4(WheelR1_BMW_X5_1) -> WheelR1_BMW_X5_1/1(WheelR1_BMW_X5_1)
  BMW_X5_1/5(WheelL1_BMW_X5_1) -> WheelL1_BMW_X5_1/1(WheelL1_BMW_X5_1)
  BMW_X5_1/6(SteeringWheel_pivot_BMW_X5_1) -> SteeringWheel_pivot_BMW_X5_1/1(SteeringWheel_pivot_BMW_X5_1)
  BMW_X5_1/7(SteeringColumn_pivot_BMW_X5_1) -> SteeringColumn_pivot_BMW_X5_1/1(SteeringColumn_pivot_BMW_X5_1)
  BMW_X5_1/8(BMW_X5_1_Brake_light_left) -> BMW_X5_1_Brake_light_left/1(BMW_X5_1_Brake_light_left)
  BMW_X5_1/9(BMW_X5_1_Brake_light_right) -> BMW_X5_1_Brake_light_right/1(BMW_X5_1_Brake_light_right)
  BMW_X5_1/10(BMW_X5_1_Indicator_front_left) -> BMW_X5_1_Indicator_front_left/1(BMW_X5_1_Indicator_front_left)
  BMW_X5_1/11(BMW_X5_1_Indicator_side_left) -> BMW_X5_1_Indicator_side_left/1(BMW_X5_1_Indicator_side_left)
  BMW_X5_1/12(BMW_X5_1_Indicator_rear_left) -> BMW_X5_1_Indicator_rear_left/1(BMW_X5_1_Indicator_rear_left)
  BMW_X5_1/13(BMW_X5_1_Indicator_front_right) -> BMW_X5_1_Indicator_front_right/1(BMW_X5_1_Indicator_front_right)
  BMW_X5_1/14(BMW_X5_1_Indicator_side_right) -> BMW_X5_1_Indicator_side_right/1(BMW_X5_1_Indicator_side_right)
  BMW_X5_1/15(BMW_X5_1_Indicator_rear_right) -> BMW_X5_1_Indicator_rear_right/1(BMW_X5_1_Indicator_rear_right)
  Sphere_1/1(STATE_Sphere_1_bus) -> STATE_Sphere_1_bus/1(STATE_Sphere_1_bus)
  SELF_Sphere_1/1(SELF_Sphere_1) -> Sphere_1/1(SELF_Sphere_1)
  Mazda_RX8_1/1(STATE_Mazda_RX8_1_bus) -> STATE_Mazda_RX8_1_bus/1(STATE_Mazda_RX8_1_bus)
  SELF_Mazda_RX8_1/1(SELF_Mazda_RX8_1) -> Mazda_RX8_1/1(SELF_Mazda_RX8_1)
  Mazda_RX8_1/2(WheelL0_Mazda_RX8_1) -> WheelL0_Mazda_RX8_1/1(WheelL0_Mazda_RX8_1)
  Mazda_RX8_1/3(WheelL1_Mazda_RX8_1) -> WheelL1_Mazda_RX8_1/1(WheelL1_Mazda_RX8_1)
  Mazda_RX8_1/4(WheelR0_Mazda_RX8_1) -> WheelR0_Mazda_RX8_1/1(WheelR0_Mazda_RX8_1)
  Mazda_RX8_1/5(WheelR1_Mazda_RX8_1) -> WheelR1_Mazda_RX8_1/1(WheelR1_Mazda_RX8_1)
  Mazda_RX8_1/6(SteeringWheel_pivot_Mazda_RX8_1) -> SteeringWheel_pivot_Mazda_RX8_1/1(SteeringWheel_pivot_Mazda_RX8_1)
  Mazda_RX8_1/7(SteeringColumn_pivot_Mazda_RX8_1) -> SteeringColumn_pivot_Mazda_RX8_1/1(SteeringColumn_pivot_Mazda_RX8_1)
  Mazda_RX8_1/8(Mazda_RX8_1_Brake_light_center) -> Mazda_RX8_1_Brake_light_center/1(Mazda_RX8_1_Brake_light_center)
  Mazda_RX8_1/9(Mazda_RX8_1_Brake_light_left) -> Mazda_RX8_1_Brake_light_left/1(Mazda_RX8_1_Brake_light_left)
  Mazda_RX8_1/10(Mazda_RX8_1_Brake_light_right) -> Mazda_RX8_1_Brake_light_right/1(Mazda_RX8_1_Brake_light_right)
  Mazda_RX8_1/11(Mazda_RX8_1_Indicator_front_left) -> Mazda_RX8_1_Indicator_front_left/1(Mazda_RX8_1_Indicator_front_left)
  Mazda_RX8_1/12(Mazda_RX8_1_Indicator_side_left) -> Mazda_RX8_1_Indicator_side_left/1(Mazda_RX8_1_Indicator_side_left)
  Mazda_RX8_1/13(Mazda_RX8_1_Indicator_rear_left) -> Mazda_RX8_1_Indicator_rear_left/1(Mazda_RX8_1_Indicator_rear_left)
  Mazda_RX8_1/14(Mazda_RX8_1_Indicator_front_right) -> Mazda_RX8_1_Indicator_front_right/1(Mazda_RX8_1_Indicator_front_right)
  Mazda_RX8_1/15(Mazda_RX8_1_Indicator_side_right) -> Mazda_RX8_1_Indicator_side_right/1(Mazda_RX8_1_Indicator_side_right)
  Mazda_RX8_1/16(Mazda_RX8_1_Indicator_rear_right) -> Mazda_RX8_1_Indicator_rear_right/1(Mazda_RX8_1_Indicator_rear_right)
  Fiat_Bravo_1/1(STATE_Fiat_Bravo_1_bus) -> STATE_Fiat_Bravo_1_bus/1(STATE_Fiat_Bravo_1_bus)
  SELF_Fiat_Bravo_1/1(SELF_Fiat_Bravo_1) -> Fiat_Bravo_1/1(SELF_Fiat_Bravo_1)
  Fiat_Bravo_1/2(WheelL0_Fiat_Bravo_1) -> WheelL0_Fiat_Bravo_1/1(WheelL0_Fiat_Bravo_1)
  Fiat_Bravo_1/3(WheelL1_Fiat_Bravo_1) -> WheelL1_Fiat_Bravo_1/1(WheelL1_Fiat_Bravo_1)
  Fiat_Bravo_1/4(WheelR0_Fiat_Bravo_1) -> WheelR0_Fiat_Bravo_1/1(WheelR0_Fiat_Bravo_1)
  Fiat_Bravo_1/5(WheelR1_Fiat_Bravo_1) -> WheelR1_Fiat_Bravo_1/1(WheelR1_Fiat_Bravo_1)
  Fiat_Bravo_1/6(SteeringWheel_pivot_Fiat_Bravo_1) -> SteeringWheel_pivot_Fiat_Bravo_1/1(SteeringWheel_pivot_Fiat_Bravo_1)
  Fiat_Bravo_1/7(SteeringColumn_pivot_Fiat_Bravo_1) -> SteeringColumn_pivot_Fiat_Bravo_1/1(SteeringColumn_pivot_Fiat_Bravo_1)
  Fiat_Bravo_1/8(Fiat_Bravo_1_Brake_light_center) -> Fiat_Bravo_1_Brake_light_center/1(Fiat_Bravo_1_Brake_light_center)
  Fiat_Bravo_1/9(Fiat_Bravo_1_Brake_light_left) -> Fiat_Bravo_1_Brake_light_left/1(Fiat_Bravo_1_Brake_light_left)
  Fiat_Bravo_1/10(Fiat_Bravo_1_Brake_light_right) -> Fiat_Bravo_1_Brake_light_right/1(Fiat_Bravo_1_Brake_light_right)
  Fiat_Bravo_1/11(Fiat_Bravo_1_Indicator_front_left) -> Fiat_Bravo_1_Indicator_front_left/1(Fiat_Bravo_1_Indicator_front_left)
  Fiat_Bravo_1/12(Fiat_Bravo_1_Indicator_side_left) -> Fiat_Bravo_1_Indicator_side_left/1(Fiat_Bravo_1_Indicator_side_left)
  Fiat_Bravo_1/13(Fiat_Bravo_1_Indicator_rear_left) -> Fiat_Bravo_1_Indicator_rear_left/1(Fiat_Bravo_1_Indicator_rear_left)
  Fiat_Bravo_1/14(Fiat_Bravo_1_Indicator_front_right) -> Fiat_Bravo_1_Indicator_front_right/1(Fiat_Bravo_1_Indicator_front_right)
  Fiat_Bravo_1/15(Fiat_Bravo_1_Indicator_side_right) -> Fiat_Bravo_1_Indicator_side_right/1(Fiat_Bravo_1_Indicator_side_right)
  Fiat_Bravo_1/16(Fiat_Bravo_1_Indicator_rear_right) -> Fiat_Bravo_1_Indicator_rear_right/1(Fiat_Bravo_1_Indicator_rear_right)
  Ford_Fiesta_1/1(STATE_Ford_Fiesta_1_bus) -> STATE_Ford_Fiesta_1_bus/1(STATE_Ford_Fiesta_1_bus)
  SELF_Ford_Fiesta_1/1(SELF_Ford_Fiesta_1) -> Ford_Fiesta_1/1(SELF_Ford_Fiesta_1)
  Ford_Fiesta_1/2(WheelL0_Ford_Fiesta_1) -> WheelL0_Ford_Fiesta_1/1(WheelL0_Ford_Fiesta_1)
  Ford_Fiesta_1/3(WheelL1_Ford_Fiesta_1) -> WheelL1_Ford_Fiesta_1/1(WheelL1_Ford_Fiesta_1)
  Ford_Fiesta_1/4(WheelR0_Ford_Fiesta_1) -> WheelR0_Ford_Fiesta_1/1(WheelR0_Ford_Fiesta_1)
  Ford_Fiesta_1/5(WheelR1_Ford_Fiesta_1) -> WheelR1_Ford_Fiesta_1/1(WheelR1_Ford_Fiesta_1)
  Ford_Fiesta_1/6(SteeringWheel_pivot_Ford_Fiesta_1) -> SteeringWheel_pivot_Ford_Fiesta_1/1(SteeringWheel_pivot_Ford_Fiesta_1)
  Ford_Fiesta_1/7(SteeringColumn_pivot_Ford_Fiesta_1) -> SteeringColumn_pivot_Ford_Fiesta_1/1(SteeringColumn_pivot_Ford_Fiesta_1)
  Ford_Fiesta_1/8(Ford_Fiesta_1_Brake_light_center) -> Ford_Fiesta_1_Brake_light_center/1(Ford_Fiesta_1_Brake_light_center)
  Ford_Fiesta_1/9(Ford_Fiesta_1_Brake_light_left) -> Ford_Fiesta_1_Brake_light_left/1(Ford_Fiesta_1_Brake_light_left)
  Ford_Fiesta_1/10(Ford_Fiesta_1_Brake_light_right) -> Ford_Fiesta_1_Brake_light_right/1(Ford_Fiesta_1_Brake_light_right)
  Ford_Fiesta_1/11(Ford_Fiesta_1_Indicator_front_left) -> Ford_Fiesta_1_Indicator_front_left/1(Ford_Fiesta_1_Indicator_front_left)
  Ford_Fiesta_1/12(Ford_Fiesta_1_Indicator_side_left) -> Ford_Fiesta_1_Indicator_side_left/1(Ford_Fiesta_1_Indicator_side_left)
  Ford_Fiesta_1/13(Ford_Fiesta_1_Indicator_rear_left) -> Ford_Fiesta_1_Indicator_rear_left/1(Ford_Fiesta_1_Indicator_rear_left)
  Ford_Fiesta_1/14(Ford_Fiesta_1_Indicator_front_right) -> Ford_Fiesta_1_Indicator_front_right/1(Ford_Fiesta_1_Indicator_front_right)
  Ford_Fiesta_1/15(Ford_Fiesta_1_Indicator_side_right) -> Ford_Fiesta_1_Indicator_side_right/1(Ford_Fiesta_1_Indicator_side_right)
  Ford_Fiesta_1/16(Ford_Fiesta_1_Indicator_rear_right) -> Ford_Fiesta_1_Indicator_rear_right/1(Ford_Fiesta_1_Indicator_rear_right)
  Honda_Pan_European_1/1(STATE_Honda_Pan_European_1_bus) -> STATE_Honda_Pan_European_1_bus/1(STATE_Honda_Pan_European_1_bus)
  SELF_Honda_Pan_European_1/1(SELF_Honda_Pan_European_1) -> Honda_Pan_European_1/1(SELF_Honda_Pan_European_1)
  Honda_Pan_European_1/2(SteeringColumn_pivot_Honda_Pan_European_1) -> SteeringColumn_pivot_Honda_Pan_European_1/1(SteeringColumn_pivot_Honda_Pan_European_1)
  Honda_Pan_European_1/3(Wheel0_Suspension_Honda_Pan_European_1) -> Wheel0_Suspension_Honda_Pan_European_1/1(Wheel0_Suspension_Honda_Pan_European_1)
  Honda_Pan_European_1/4(Wheel0_Honda_Pan_European_1) -> Wheel0_Honda_Pan_European_1/1(Wheel0_Honda_Pan_European_1)
  Honda_Pan_European_1/5(Wheel1_Suspension_Honda_Pan_European_1) -> Wheel1_Suspension_Honda_Pan_European_1/1(Wheel1_Suspension_Honda_Pan_European_1)
  Honda_Pan_European_1/6(Wheel1_Honda_Pan_European_1) -> Wheel1_Honda_Pan_European_1/1(Wheel1_Honda_Pan_European_1)
  Honda_Pan_European_1/7(Honda_Pan_European_1_Brake_light_center) -> Honda_Pan_European_1_Brake_light_center/1(Honda_Pan_European_1_Brake_light_center)
  Honda_Pan_European_1/8(Honda_Pan_European_1_Indicator_front_left) -> Honda_Pan_European_1_Indicator_front_left/1(Honda_Pan_European_1_Indicator_front_left)
  Honda_Pan_European_1/9(Honda_Pan_European_1_Indicator_front_right) -> Honda_Pan_European_1_Indicator_front_right/1(Honda_Pan_European_1_Indicator_front_right)
  Honda_Pan_European_1/10(Honda_Pan_European_1_Indicator_rear_left) -> Honda_Pan_European_1_Indicator_rear_left/1(Honda_Pan_European_1_Indicator_rear_left)
  Honda_Pan_European_1/11(Honda_Pan_European_1_Indicator_rear_right) -> Honda_Pan_European_1_Indicator_rear_right/1(Honda_Pan_European_1_Indicator_rear_right)
  Toyota_Yaris_1/1(STATE_Toyota_Yaris_1_bus) -> STATE_Toyota_Yaris_1_bus/1(STATE_Toyota_Yaris_1_bus)
  SELF_Toyota_Yaris_1/1(SELF_Toyota_Yaris_1) -> Toyota_Yaris_1/1(SELF_Toyota_Yaris_1)
  Toyota_Yaris_1/2(WheelL0_Toyota_Yaris_1) -> WheelL0_Toyota_Yaris_1/1(WheelL0_Toyota_Yaris_1)
  Toyota_Yaris_1/3(WheelL1_Toyota_Yaris_1) -> WheelL1_Toyota_Yaris_1/1(WheelL1_Toyota_Yaris_1)
  Toyota_Yaris_1/4(WheelR0_Toyota_Yaris_1) -> WheelR0_Toyota_Yaris_1/1(WheelR0_Toyota_Yaris_1)
  Toyota_Yaris_1/5(WheelR1_Toyota_Yaris_1) -> WheelR1_Toyota_Yaris_1/1(WheelR1_Toyota_Yaris_1)
  Toyota_Yaris_1/6(SteeringWheel_pivot_Toyota_Yaris_1) -> SteeringWheel_pivot_Toyota_Yaris_1/1(SteeringWheel_pivot_Toyota_Yaris_1)
  Toyota_Yaris_1/7(SteeringColumn_pivot_Toyota_Yaris_1) -> SteeringColumn_pivot_Toyota_Yaris_1/1(SteeringColumn_pivot_Toyota_Yaris_1)
  Toyota_Yaris_1/8(Toyota_Yaris_1_Brake_light_left) -> Toyota_Yaris_1_Brake_light_left/1(Toyota_Yaris_1_Brake_light_left)
  Toyota_Yaris_1/9(Toyota_Yaris_1_Brake_light_right) -> Toyota_Yaris_1_Brake_light_right/1(Toyota_Yaris_1_Brake_light_right)
  Toyota_Yaris_1/10(Toyota_Yaris_1_Indicator_front_left) -> Toyota_Yaris_1_Indicator_front_left/1(Toyota_Yaris_1_Indicator_front_left)
  Toyota_Yaris_1/11(Toyota_Yaris_1_Indicator_side_left) -> Toyota_Yaris_1_Indicator_side_left/1(Toyota_Yaris_1_Indicator_side_left)
  Toyota_Yaris_1/12(Toyota_Yaris_1_Indicator_rear_left) -> Toyota_Yaris_1_Indicator_rear_left/1(Toyota_Yaris_1_Indicator_rear_left)
  Toyota_Yaris_1/13(Toyota_Yaris_1_Indicator_front_right) -> Toyota_Yaris_1_Indicator_front_right/1(Toyota_Yaris_1_Indicator_front_right)
  Toyota_Yaris_1/14(Toyota_Yaris_1_Indicator_side_right) -> Toyota_Yaris_1_Indicator_side_right/1(Toyota_Yaris_1_Indicator_side_right)
  Toyota_Yaris_1/15(Toyota_Yaris_1_Indicator_rear_right) -> Toyota_Yaris_1_Indicator_rear_right/1(Toyota_Yaris_1_Indicator_rear_right)
  HighwayOverhang_1/1(VISUMatrixSign_HighwayOverhang_1) -> VISUMatrixSign_HighwayOverhang_1/1(VISUMatrixSign_HighwayOverhang_1)
  HighwayOverhang_1/2(VISUMatrixSignLights_HighwayOverhang_1) -> VISUMatrixSignLights_HighwayOverhang_1/1(VISUMatrixSignLights_HighwayOverhang_1)
  HighwayOverhang_2/1(VISUMatrixSign_HighwayOverhang_2) -> VISUMatrixSign_HighwayOverhang_2/1(VISUMatrixSign_HighwayOverhang_2)
  HighwayOverhang_2/2(VISUMatrixSignLights_HighwayOverhang_2) -> VISUMatrixSignLights_HighwayOverhang_2/1(VISUMatrixSignLights_HighwayOverhang_2)
  HighwayOverhang_3/1(VISUMatrixSign_HighwayOverhang_3) -> VISUMatrixSign_HighwayOverhang_3/1(VISUMatrixSign_HighwayOverhang_3)
  HighwayOverhang_4/1(VISUMatrixSign_HighwayOverhang_4) -> VISUMatrixSign_HighwayOverhang_4/1(VISUMatrixSign_HighwayOverhang_4)
  HighwayOverhang_5/1(VISUMatrixSign_HighwayOverhang_5) -> VISUMatrixSign_HighwayOverhang_5/1(VISUMatrixSign_HighwayOverhang_5)
  HighwayOverhang_6/1(VISUMatrixSign_HighwayOverhang_6) -> VISUMatrixSign_HighwayOverhang_6/1(VISUMatrixSign_HighwayOverhang_6)
  HighwayOverhang_7/1(VISUMatrixSign_HighwayOverhang_7) -> VISUMatrixSign_HighwayOverhang_7/1(VISUMatrixSign_HighwayOverhang_7)
  HighwayOverhang_8/1(VISUMatrixSign_HighwayOverhang_8) -> VISUMatrixSign_HighwayOverhang_8/1(VISUMatrixSign_HighwayOverhang_8)
  HighwayOverhang_9/1(VISUMatrixSign_HighwayOverhang_9) -> VISUMatrixSign_HighwayOverhang_9/1(VISUMatrixSign_HighwayOverhang_9)
  HighwayOverhang_10/1(VISUMatrixSign_HighwayOverhang_10) -> VISUMatrixSign_HighwayOverhang_10/1(VISUMatrixSign_HighwayOverhang_10)
  HighwayOverhang_11/1(VISUMatrixSign_HighwayOverhang_11) -> VISUMatrixSign_HighwayOverhang_11/1(VISUMatrixSign_HighwayOverhang_11)
  HighwayOverhang_11/2(VISUMatrixSignLights_HighwayOverhang_11) -> VISUMatrixSignLights_HighwayOverhang_11/1(VISUMatrixSignLights_HighwayOverhang_11)
  HighwayOverhang_12/1(VISUMatrixSign_HighwayOverhang_12) -> VISUMatrixSign_HighwayOverhang_12/1(VISUMatrixSign_HighwayOverhang_12)
  HighwayOverhang_12/2(VISUMatrixSignLights_HighwayOverhang_12) -> VISUMatrixSignLights_HighwayOverhang_12/1(VISUMatrixSignLights_HighwayOverhang_12)
